simulink model "IEEE123bus_v2019b_Phasor_DPL_ZIPload"  (R2019b)
settings: Solver=VariableStepAuto  StartTime=0.0  StopTime=100  FixedStep=Ts  RelTol=1e-3
InitFcn:
  | a=1; % Loading Factor
  | Ts=0.1;% For Delay Blocks in Voltage Regulator Controls
  | 
  | % Simulation data for the IEEE 123 Node Test Feeder model
  | mi2km = 1.60934;%  miles to km conversion
  | ft2km = 0.0003048; % feet to km conversion
  | ms2F = 1*1e-6/(2*pi*60);% microsiemens to Farads conversion
  | 
  | %% Configuration 1
  | % Series Resitance and Reactance - ohm/mile
  | R_1 = [0.4576 0.1560 0.1535;0.1560 0.4666 0.1580;0.1535 0.1580 0.4615];
  | X_1 = [1.0780 0.5017 0.3849;0.5017 1.0482 0.4236;0.3849 0.4236 1.0651];
  | % charging susceptance - microsiemens/mile
  | B_1 = [5.6765 -1.8319 -0.6982;-1.8319 5.9809 -1.1645;-0.6982 -1.1645 5.3971];
  | 
  | R_1 = R_1/mi2km;
  | L_1 = (X_1/(2*pi*60))/mi2km;
  | C_1 =(B_1*ms2F)/mi2km;
  | 
  | %% Configuration 2 - series reactance - ohm/mile
  | R_2 = [0.4666 0.1580 0.1560;0.1580 0.4615 0.1535;0.1560 0.1535 0.4576];
  | X_2 = [1.0482 0.4236 0.5017;0.4236 1.0651 0.3849;0.5017 0.3849 1.0780];
  | % charging susceptance - microsiemens/mile
  | B_2 = [5.9809 -1.1645 -1.8319;-1.1645 5.3971 -0.6982;-1.8319 -0.6982 5.6765];
  | 
  | R_2 = R_2/mi2km;
  | L_2 = (X_2/(2*pi*60))/mi2km;
  | C_2 =(B_2*ms2F)/mi2km;
  | 
  | %% Configuration 3 - series reactance - ohm/mile
  | R_3 = [0.4615 0.1535 0.1580;0.1535 0.4576 0.1560;0.1580 0.1560 0.4666];
  | X_3 = [1.0651 0.3849 0.4236;0.3849 1.0780 0.5017;0.4236 0.5017 1.0482];
  | % charging susceptance - microsiemens/mile
  | B_3 = [5.3971 -0.6982 -1.1645;-0.6982 5.6765 -1.8319; -1.1645 -1.8319 5.9809];
  | 
  | R_3 = R_3/mi2km;
  | L_3 = (X_3/(2*pi*60))/mi2km;
  | C_3 =(B_3*ms2F)/mi2km;
  | 
  | %% Configuration 4 - series reactance - ohm/mile
  | R_4 = [0.4615 0.1580 0.1535;0.1580 0.4666 0.1560;0.1535 0.1560 0.4576];
  | X_4 = [1.0651 0.4236 0.3849;0.4236 1.0482 0.5017;0.3849 0.5017 1.0780];
  | % charging susceptance - microsiemens/mile
  | B_4 = [5.3971 -1.1645 -0.6982;-1.1645 5.9809 -1.8319;-0.6982 -1.8319 5.6765];
  | 
  | R_4 = R_4/mi2km;
  | L_4 = (X_4/(2*pi*60))/mi2km;
  | C_4 =(B_4*ms2F)/mi2km;
  | 
  | %% Configuration 5 - series reactance - ohm/mile
  | R_5 = [0.4666 0.1560 0.1580;0.1560 0.4576 0.1535;0.1580 0.1535 0.4615];
  | X_5 = [1.0482 0.5017 0.4236;0.5017 1.0780 0.3849;0.4236 0.3849 1.0651];
  | % charging susceptance - microsiemens/mile
  | B_5 = [5.9809 -1.8319 -1.1645;-1.8319 5.6765 -0.6982;-1.1645 -0.6982 5.3971];
  | 
  | R_5 = R_5/mi2km;
  | L_5 = (X_5/(2*pi*60))/mi2km;
  | C_5 =(B_5*ms2F)/mi2km;
  | 
  | %% Configuration 6 - series reactance - ohm/mile
  | R_6 = [0.4576 0.1535 0.1560;0.1535 0.4615 0.1580;0.1560 0.1580 0.4666];
  | X_6 = [1.0780 0.3849 0.5017;0.3849 1.0651 0.4236;0.5017 0.4236 1.0482];
  | % charging susceptance - microsiemens/mile
  | B_6 = [5.6765 -0.6982 -1.8319;-0.6982 5.3971 -1.1645;-1.8319 -1.1645 5.9809];
  | 
  | R_6 = R_6/mi2km;
  | L_6 = (X_6/(2*pi*60))/mi2km;
  | C_6 =(B_6*ms2F)/mi2km;
  | 
  | %% Configuration 7 - series reactance - ohm/mile
  | R_7 = [0.4576 0.0000 0.1535;0.0000 0.0000 0.0000;0.1535 0.0000 0.4615];
  | X_7 = [1.0780 0.0000 0.3849;0.0000 0.0000 0.0000;0.3849 0.0000 1.0651];
  | % charging susceptance - microsiemens/mile
  | B_7 = [5.1154 0.0000 -1.0549;0.0000 0.0000 0.0000;-1.0549 0.0000 5.1704];
  | 
  | R_7 = R_7/mi2km;
  | L_7 = (X_7/(2*pi*60))/mi2km;
  | C_7 =(B_7*ms2F)/mi2km;
  | 
  | %% Configuration 8 - series reactance - ohm/mile
  | R_8 = [0.4576 0.1535 0.0000;0.1535 0.4615 0.0000;0.0000 0.0000 0.0000];
  | X_8 = [1.0780 0.3849 0.0000;0.3849 1.0651 0.0000;0.0000 0.0000 0.0000];
  | % charging susceptance - microsiemens/mile
  | B_8 = [5.1154 -1.0549 0.0000;-1.0549 5.1704 0.0000;0.0000 0.0000 0.0000];
  | 
  | R_8 = R_8/mi2km;
  | L_8 = (X_8/(2*pi*60))/mi2km;
  | C_8 =(B_8*ms2F)/mi2km;
  | 
  | %% Configuration 9 - series reactance - ohm/mile
  | R_9 = [1.3292 0 0;0 0 0;0 0 0];
  | X_9 = [1.3475 0 0;0 0 0;0 0 0];
  | % charging susceptance - microsiemens/mile
  | B_9 = [4.5193 0 0;0 0 0;0 0 0];
  | 
  | R_9 = R_9/mi2km;
  | L_9 = (X_9/(2*pi*60))/mi2km;
  | C_9 =(B_9*ms2F)/mi2km;
  | 
  | %% Configuration 10- series reactance - ohm/mile
  | R_10 = [0 0 0;0 1.3292 0;0 0 0];
  | X_10 = [0 0 0;0 1.3475 0;0 0 0];
  | % charging susceptance - microsiemens/mile
  | B_10 = [0 0 0;0 4.5193 0;0 0 0];
  | 
  | R_10 = R_10/mi2km;
  | L_10 = (X_10/(2*pi*60))/mi2km;
  | C_10 =(B_10*ms2F)/mi2km;
  | 
  | %% Configuration 11 - series reactance - ohm/mile
  | R_11 = [0 0 0;0 0 0;0 0 1.3292];
  | X_11 = [0 0 0;0 0 0;0 0 1.3475];
  | % charging susceptance - microsiemens/mile
  | B_11 = [0 0 0;0 0 0;0 0 4.5193];
  | 
  | R_11 = R_11/mi2km;
  | L_11 = (X_11/(2*pi*60))/mi2km;
  | C_11 =(B_11*ms2F)/mi2km;
  | 
  | %% Configuration 12 - series reactance - ohm/mile
  | R_12 = [1.5209 0.5198 0.4924;0.5198 1.5329 0.5198;0.4924 0.5198 1.5209];
  | X_12 = [0.7521 0.2775 0.2157;0.2775 0.7162 0.2775;0.2157 0.2775 0.7521];
  | % charging susceptance - microsiemens/mile
  | B_12 = [67.2242 0.0000 0.0000;0.0000 67.2242 0.0000;0.0000 0.0000 67.2242];
  | 
  | R_12 = R_12/mi2km;
  | L_12 = (X_12/(2*pi*60))/mi2km;
  | C_12 =(B_12*ms2F)/mi2km;
undefined symbols (not defined in the file or in its folder): D1, Delta, find_system, j
libraries: powerlib x886, powerlib_meascontrol x31
(part 1 of 12)
settings Model: ARTEMISmethode_block_infos=$$__separator__$$pi123variableloadwith3PV/ARTEMIS Guide$$__separator__$$  Creator=Arun  LastModifiedBy=USARSUR
settings DataIOCC: ReturnWorkspaceOutputs=off
settings DebuggingCC: UnconnectedInputMsg=none  UnconnectedOutputMsg=none  UnconnectedLineMsg=none  ArithmeticOperatorsInVariantConditions=warning
settings SFSimCC: SimUseLocalCustomCode=off  CustomCodeUndefinedFunction=UseInterfaceOnly
settings RTWCC: RTWUseLocalCustomCode=off
settings CodeAppCC: StateflowObjectComments=on
settings SimscapeCC: SimscapeNormalizeSystem=off

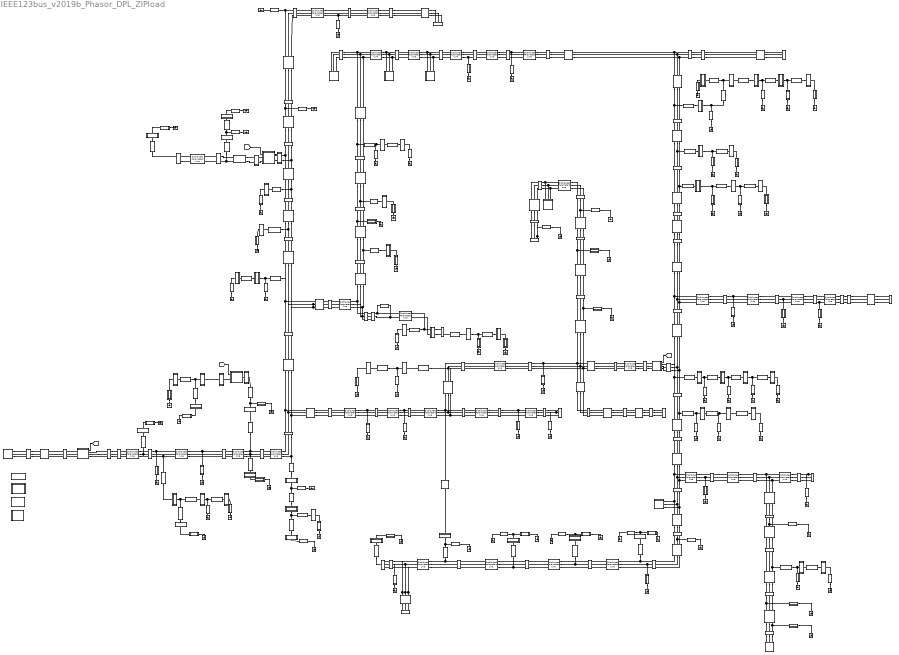
== system IEEE123bus_v2019b_Phasor_DPL_ZIPload ==
  note: Please consider citing following papers if the model was useful for your research
      |
      | A. Suresh, R. Bisht and S. Kamalasadan, "A Coordinated Control Architecture With Inverter-Based Resources and Legacy
      | Controllers of Power Distribution System for Voltage Profile Balance," in IEEE Transactions on Industry Applications, vol. 58,
      | no. 5, pp. 6701-6712, Sept.-Oct. 2022, doi: 10.1109/TIA.2022.3183030.
      |
      | A. Suresh, R. Bisht and S. Kamalasadan, "ADMM Based LQR for Voltage Regulation Using Distributed Energy Resources,"
      | 2020 IEEE International Conference on Power Electronics, Drives and Energy Systems (PEDES), 2020, pp. 1-6,
      | doi: 10.1109/PEDES49360.2020.9379625.
  note: Model Developed by
      | Arun Suresh, Dr. Sukumar Kamalasadan,
      | University of North Carolina, Charlotte
  1 : powerlib/Measurements/Three-Phase V-I Measurement  VoltageMeasurement=phase-to-ground  SetLabelV=on  LabelV=V1  Vpu=off  VpuLL=off  CurrentMeasurement=no  SetLabelI=on  LabelI=I800  Ipu=off  Pbase=100e6  Vbase=24900  OutputType=Complex  PhasorSimulation=on  PSBequivalent=0
      settings: SourceProductName=Simscape Electrical
  1 Y PQ : Subsystem  mask(Single Phase ZIP Load){Vnom=1.0*2401.78, fnom=60, Pnom=40e3*a, Qnom=20e3*a, LoadType=constant P, Vlim=0.7}
      mask prompts: Vnom "Nominal Voltage Vn (Vrms)"; fnom "Nominal Frequency fn (Hz)"; Pnom "Nominal Active power (W)"; Qnom "Nominal Reactive power (VAR)"; LoadType "Load Type"; Vlim "Minimum voltage (pu)"
      mask help:
      | Notes:
      | Single Phase ZIP load model which gets converted to constant Z type if the voltage becomes lower than the Minimum Voltage.
      mask TypeOptions LoadType: Constant Z | constant I | constant P
      mask DialogControl ParameterTabVar0 Prompt: Parameters
      mask DialogControl ParameterTabVar1 Prompt: Type
      mask Display:
      | color('red');
      | A=[-210,-180,-170,-160,-147,-140,-130,-120,-110,-80,-50,-49,-45,-39,-33,-26,-21,-18,-17,-19,-22,-22,-26,-27,-25,-22,-16,-9,-3,2,6,6,4,1,1,-3,-4,-2,2,7,14,20,26,29,30,28,24,24,21,20,21,25,31,37,44,49,50,50,80];
      | B=[-41.5,-41.5,-63,-20,-63,-20,-63,-20,-41.5,-41.5,-41.5,-34,-26,-21,-20,-22,-28,-37,-47,-57,-63,-63,-54,-44,-34,-26,-21,-20,-22,-28,-37,-47,-57,-63,-63,-54,-44,-34,-26,-21,-20,-22,-28,-37,-47,-57,-63,-63,-54,-44,-34,-26,-21,-20,-22,-28,-37,-41.50,-41.5];
      | plot(A,B);
      | color('black');
      | port_label('LConn', 1, '+')
  1-2 10 : powerlib/Elements/Distributed Parameters Line  Phases=1  Frequency=60  Resistance=R_10(2,2)  Inductance=L_10(2,2)  Capacitance=C_10(2,2)  Length=175*ft2km  x1=[3403.40407583669;376.991118430775;-2.09535227015144]  x2=[3403.40393728209;376.991118430775;-2.09535231811345]  x3=[6.22904140851351;376.991118430775;-2.09543411070126]  x4=[6.2358477770861;376.991118430775;-2.09535231481402]  x5=2.16957196133287e-07  V1=[2.049e+04;377;-2.115]  V2=[2.048e+04;377;-2.115]  I1=[33.62;377;-2.106]  I2=[35.2;377;-2.126]  nHarmo=1  Measurements=None
      settings: SourceProductName=Simscape Electrical
  1-3 11 : powerlib/Elements/Distributed Parameters Line  Phases=1  Frequency=60  Resistance=R_11(3,3)  Inductance=L_11(3,3)  Capacitance=C_11(3,3)  Length=250*ft2km  x1=[3404.23228446094;376.991118430775;2.09338339619212]  x2=[3404.23180903077;376.991118430775;2.09338315630066]  x3=[6.22358820978929;376.991118430775;2.09290352483269]  x4=[6.24401143477824;376.991118430775;2.09374480200052]  x5=3.09938851618982e-07  V1=[2.049e+04;377;-2.115]  V2=[2.048e+04;377;-2.115]  I1=[33.62;377;-2.106]  I2=[35.2;377;-2.126]  nHarmo=1  Measurements=None
      settings: SourceProductName=Simscape Electrical
  1-7 1 : powerlib/Elements/Distributed Parameters Line  Phases=3  Frequency=60  Resistance=R_1  Inductance=L_1  Capacitance=C_1  Length=300*ft2km  x1=[436.800297543745 4167.29457653455 4166.80094747361;376.991118430775 376.991118430775 376.991118430775;1.69106599673736 -2.40312878788664 2.3092308326774]  x2=[437.061191479492 4173.08837477824 4174.13245807205;376.991118430775 376.991118430775 376.991118430775;1.69067039189404 -2.40392213512409 2.30843926486521]  x3=[2.63602464413822 185.698581223299 185.612678797795;376.991118430775 376.991118430775 376.991118430775;0.131396490934745 2.37819332141936 0.79306646276384]  x4=[2.86335918238174 186.149188672012 185.887033927544;376.991118430775 376.991118430775 376.991118430775;2.8602728168382 -0.931024482265744 -2.48097001414768]  x5=3.76244991844366e-07  V1=ones(3,3)  V2=ones(3,3)  I1=ones(3,3)  I2=ones(3,3)  nHarmo=1  Measurements=None
      settings: SourceProductName=Simscape Electrical
  10 : Subsystem
  10 Y I : Subsystem  mask(Single Phase ZIP Load){Vnom=1.0*2401.78, fnom=60, Pnom=20e3*a, Qnom=10e3*a, LoadType=constant I, Vlim=0.7}
      mask prompts: Vnom "Nominal Voltage Vn (Vrms)"; fnom "Nominal Frequency fn (Hz)"; Pnom "Nominal Active power (W)"; Qnom "Nominal Reactive power (VAR)"; LoadType "Load Type"; Vlim "Minimum voltage (pu)"
      mask help:
      | Notes:
      | Single Phase ZIP load model which gets converted to constant Z type if the voltage becomes lower than the Minimum Voltage.
      mask TypeOptions LoadType: Constant Z | constant I | constant P
      mask DialogControl ParameterTabVar0 Prompt: Parameters
      mask DialogControl ParameterTabVar1 Prompt: Type
      mask Display:
      | color('red');
      | A=[-210,-180,-170,-160,-147,-140,-130,-120,-110,-80,-50,-49,-45,-39,-33,-26,-21,-18,-17,-19,-22,-22,-26,-27,-25,-22,-16,-9,-3,2,6,6,4,1,1,-3,-4,-2,2,7,14,20,26,29,30,28,24,24,21,20,21,25,31,37,44,49,50,50,80];
      | B=[-41.5,-41.5,-63,-20,-63,-20,-63,-20,-41.5,-41.5,-41.5,-34,-26,-21,-20,-22,-28,-37,-47,-57,-63,-63,-54,-44,-34,-26,-21,-20,-22,-28,-37,-47,-57,-63,-63,-54,-44,-34,-26,-21,-20,-22,-28,-37,-47,-57,-63,-63,-54,-44,-34,-26,-21,-20,-22,-28,-37,-41.50,-41.5];
      | plot(A,B);
      | color('black');
      | port_label('LConn', 1, '+')
  100 : powerlib/Measurements/Three-Phase V-I Measurement  VoltageMeasurement=phase-to-ground  SetLabelV=on  LabelV=V100  Vpu=off  VpuLL=off  CurrentMeasurement=no  SetLabelI=on  LabelI=I65  Ipu=off  Pbase=100e6  Vbase=24900  OutputType=Complex  PhasorSimulation=on  PSBequivalent=0
      settings: SourceProductName=Simscape Electrical
  100 Y Z : Subsystem  mask(Single Phase ZIP Load){Vnom=1.0*2401.78, fnom=60, Pnom=40e3*a, Qnom=20e3*a, LoadType=Constant Z, Vlim=0.7}
      mask prompts: Vnom "Nominal Voltage Vn (Vrms)"; fnom "Nominal Frequency fn (Hz)"; Pnom "Nominal Active power (W)"; Qnom "Nominal Reactive power (VAR)"; LoadType "Load Type"; Vlim "Minimum voltage (pu)"
      mask help:
      | Notes:
      | Single Phase ZIP load model which gets converted to constant Z type if the voltage becomes lower than the Minimum Voltage.
      mask TypeOptions LoadType: Constant Z | constant I | constant P
      mask DialogControl ParameterTabVar0 Prompt: Parameters
      mask DialogControl ParameterTabVar1 Prompt: Type
      mask Display:
      | color('red');
      | A=[-210,-180,-170,-160,-147,-140,-130,-120,-110,-80,-50,-49,-45,-39,-33,-26,-21,-18,-17,-19,-22,-22,-26,-27,-25,-22,-16,-9,-3,2,6,6,4,1,1,-3,-4,-2,2,7,14,20,26,29,30,28,24,24,21,20,21,25,31,37,44,49,50,50,80];
      | B=[-41.5,-41.5,-63,-20,-63,-20,-63,-20,-41.5,-41.5,-41.5,-34,-26,-21,-20,-22,-28,-37,-47,-57,-63,-63,-54,-44,-34,-26,-21,-20,-22,-28,-37,-47,-57,-63,-63,-54,-44,-34,-26,-21,-20,-22,-28,-37,-47,-57,-63,-63,-54,-44,-34,-26,-21,-20,-22,-28,-37,-41.50,-41.5];
      | plot(A,B);
      | color('black');
      | port_label('LConn', 1, '+')
  100-450 3 : powerlib/Elements/Distributed Parameters Line  Phases=3  Frequency=60  Resistance=R_3  Inductance=L_3  Capacitance=C_3  Length=800*ft2km  x1=[443.373552146088 4232.26022753008 4232.1634537403;376.991118430775 376.991118430775 376.991118430775;-0.417224791555343 0.205878059890174 1.77874707649804]  x2=[443.373583862276 4232.26043412699 4232.16366214147;376.991118430775 376.991118430775 376.991118430775;-0.417224820253187 0.20587803856342 1.77874704932021]  x3=[0.582709365484829 12.4738244359709 15.7961847761454;376.991118430775 376.991118430775 376.991118430775;-0.417603048631578 0.205565591892628 1.77843324057499]  x4=[0.582709365503137 12.4738244359882 15.7961847761854;376.991118430775 376.991118430775 376.991118430775;-0.417224820241726 0.205878038563425 1.7787470493196]  x5=1.00331997825164e-06  V1=ones(3,3)  V2=ones(3,3)  I1=ones(3,3)  I2=ones(3,3)  nHarmo=1  Measurements=None
      settings: SourceProductName=Simscape Electrical
  101 : powerlib/Measurements/Three-Phase V-I Measurement  VoltageMeasurement=phase-to-ground  SetLabelV=on  LabelV=V101  Vpu=off  VpuLL=off  CurrentMeasurement=no  SetLabelI=on  LabelI=I65  Ipu=off  Pbase=100e6  Vbase=24900  OutputType=Complex  PhasorSimulation=on  PSBequivalent=0
      settings: SourceProductName=Simscape Electrical
  101-102 11 : powerlib/Elements/Distributed Parameters Line  Phases=1  Frequency=60  Resistance=R_11(3,3)  Inductance=L_11(3,3)  Capacitance=C_11(3,3)  Length=225*ft2km  x1=[3457.92797170476;376.991118430775;2.08694980209931]  x2=[3457.92757743413;376.991118430775;2.08694957468531]  x3=[6.32180933144979;376.991118430775;2.08636460802156]  x4=[6.3425547416883;376.991118430775;2.08742786454813]  x5=2.78944966457084e-07  V1=[2.049e+04;377;-2.115]  V2=[2.048e+04;377;-2.115]  I1=[33.62;377;-2.106]  I2=[35.2;377;-2.126]  nHarmo=1  Measurements=None
      settings: SourceProductName=Simscape Electrical
  101-105 3 : powerlib/Elements/Distributed Parameters Line  Phases=3  Frequency=60  Resistance=R_3  Inductance=L_3  Capacitance=C_3  Length=275*ft2km  x1=[443.373660115841 4232.25950788553 4232.16299468928;376.991118430775 376.991118430775 376.991118430775;-0.416978675467481 0.206083103238666 1.77895313392089]  x2=[443.374129264306 4232.25962050144 4232.16326999734;376.991118430775 376.991118430775 376.991118430775;-0.416979795125428 0.206082912265049 1.77895300387884]  x3=[0.580098762037406 12.4571733375896 15.786970190557;376.991118430775 376.991118430775 376.991118430775;-0.427075702485888 0.20516777463084 1.77792629805874]  x4=[0.585465938762827 12.4921559124847 15.8081037031614;376.991118430775 376.991118430775 376.991118430775;-0.407104755765716 0.206888419808551 1.77987066114847]  x5=3.44891242524002e-07  V1=ones(3,3)  V2=ones(3,3)  I1=ones(3,3)  I2=ones(3,3)  nHarmo=1  Measurements=None
      settings: SourceProductName=Simscape Electrical
  102 : Subsystem
  102 Y PQ : Subsystem  mask(Single Phase ZIP Load){Vnom=1.0*2401.78, fnom=60, Pnom=20e3*a, Qnom=10e3*a, LoadType=constant P, Vlim=0.7}
      mask prompts: Vnom "Nominal Voltage Vn (Vrms)"; fnom "Nominal Frequency fn (Hz)"; Pnom "Nominal Active power (W)"; Qnom "Nominal Reactive power (VAR)"; LoadType "Load Type"; Vlim "Minimum voltage (pu)"
      mask help:
      | Notes:
      | Single Phase ZIP load model which gets converted to constant Z type if the voltage becomes lower than the Minimum Voltage.
      mask TypeOptions LoadType: Constant Z | constant I | constant P
      mask DialogControl ParameterTabVar0 Prompt: Parameters
      mask DialogControl ParameterTabVar1 Prompt: Type
      mask Display:
      | color('red');
      | A=[-210,-180,-170,-160,-147,-140,-130,-120,-110,-80,-50,-49,-45,-39,-33,-26,-21,-18,-17,-19,-22,-22,-26,-27,-25,-22,-16,-9,-3,2,6,6,4,1,1,-3,-4,-2,2,7,14,20,26,29,30,28,24,24,21,20,21,25,31,37,44,49,50,50,80];
      | B=[-41.5,-41.5,-63,-20,-63,-20,-63,-20,-41.5,-41.5,-41.5,-34,-26,-21,-20,-22,-28,-37,-47,-57,-63,-63,-54,-44,-34,-26,-21,-20,-22,-28,-37,-47,-57,-63,-63,-54,-44,-34,-26,-21,-20,-22,-28,-37,-47,-57,-63,-63,-54,-44,-34,-26,-21,-20,-22,-28,-37,-41.50,-41.5];
      | plot(A,B);
      | color('black');
      | port_label('LConn', 1, '+')
  102-103 11 : powerlib/Elements/Distributed Parameters Line  Phases=1  Frequency=60  Resistance=R_11(3,3)  Inductance=L_11(3,3)  Capacitance=C_11(3,3)  Length=325*ft2km  x1=[3457.92757743413;376.991118430775;2.08690283700759]  x2=[3457.92722333804;376.991118430775;2.08690261072161]  x3=[6.32504721964269;376.991118430775;2.08642323448268]  x4=[6.33887685523373;376.991118430775;2.08722942969897]  x5=4.02920507104677e-07  V1=[2.049e+04;377;-2.115]  V2=[2.048e+04;377;-2.115]  I1=[33.62;377;-2.106]  I2=[35.2;377;-2.126]  nHarmo=1  Measurements=None
      settings: SourceProductName=Simscape Electrical
  103 : Subsystem
  103 Y PQ : Subsystem  mask(Single Phase ZIP Load){Vnom=1.0*2401.78, fnom=60, Pnom=40e3*a, Qnom=20e3*a, LoadType=constant P, Vlim=0.7}
      mask prompts: Vnom "Nominal Voltage Vn (Vrms)"; fnom "Nominal Frequency fn (Hz)"; Pnom "Nominal Active power (W)"; Qnom "Nominal Reactive power (VAR)"; LoadType "Load Type"; Vlim "Minimum voltage (pu)"
      mask help:
      | Notes:
      | Single Phase ZIP load model which gets converted to constant Z type if the voltage becomes lower than the Minimum Voltage.
      mask TypeOptions LoadType: Constant Z | constant I | constant P
      mask DialogControl ParameterTabVar0 Prompt: Parameters
      mask DialogControl ParameterTabVar1 Prompt: Type
      mask Display:
      | color('red');
      | A=[-210,-180,-170,-160,-147,-140,-130,-120,-110,-80,-50,-49,-45,-39,-33,-26,-21,-18,-17,-19,-22,-22,-26,-27,-25,-22,-16,-9,-3,2,6,6,4,1,1,-3,-4,-2,2,7,14,20,26,29,30,28,24,24,21,20,21,25,31,37,44,49,50,50,80];
      | B=[-41.5,-41.5,-63,-20,-63,-20,-63,-20,-41.5,-41.5,-41.5,-34,-26,-21,-20,-22,-28,-37,-47,-57,-63,-63,-54,-44,-34,-26,-21,-20,-22,-28,-37,-47,-57,-63,-63,-54,-44,-34,-26,-21,-20,-22,-28,-37,-47,-57,-63,-63,-54,-44,-34,-26,-21,-20,-22,-28,-37,-41.50,-41.5];
      | plot(A,B);
      | color('black');
      | port_label('LConn', 1, '+')
  103-104 11 : powerlib/Elements/Distributed Parameters Line  Phases=1  Frequency=60  Resistance=R_11(3,3)  Inductance=L_11(3,3)  Capacitance=C_11(3,3)  Length=700*ft2km  x1=[3457.92722333804;376.991118430775;2.08672734443013]  x2=[3457.92679904314;376.991118430775;2.08672711299265]  x3=[6.32768318900497;376.991118430775;2.08639997569265]  x4=[6.33459681116843;376.991118430775;2.08672711297322]  x5=8.6782878453315e-07  V1=[2.049e+04;377;-2.115]  V2=[2.048e+04;377;-2.115]  I1=[33.62;377;-2.106]  I2=[35.2;377;-2.126]  nHarmo=1  Measurements=None
      settings: SourceProductName=Simscape Electrical
  104 : Subsystem
  104 Y PQ : Subsystem  mask(Single Phase ZIP Load){Vnom=1.0*2401.78, fnom=60, Pnom=40e3*a, Qnom=20e3*a, LoadType=constant P, Vlim=0.7}
      mask prompts: Vnom "Nominal Voltage Vn (Vrms)"; fnom "Nominal Frequency fn (Hz)"; Pnom "Nominal Active power (W)"; Qnom "Nominal Reactive power (VAR)"; LoadType "Load Type"; Vlim "Minimum voltage (pu)"
      mask help:
      | Notes:
      | Single Phase ZIP load model which gets converted to constant Z type if the voltage becomes lower than the Minimum Voltage.
      mask TypeOptions LoadType: Constant Z | constant I | constant P
      mask DialogControl ParameterTabVar0 Prompt: Parameters
      mask DialogControl ParameterTabVar1 Prompt: Type
      mask Display:
      | color('red');
      | A=[-210,-180,-170,-160,-147,-140,-130,-120,-110,-80,-50,-49,-45,-39,-33,-26,-21,-18,-17,-19,-22,-22,-26,-27,-25,-22,-16,-9,-3,2,6,6,4,1,1,-3,-4,-2,2,7,14,20,26,29,30,28,24,24,21,20,21,25,31,37,44,49,50,50,80];
      | B=[-41.5,-41.5,-63,-20,-63,-20,-63,-20,-41.5,-41.5,-41.5,-34,-26,-21,-20,-22,-28,-37,-47,-57,-63,-63,-54,-44,-34,-26,-21,-20,-22,-28,-37,-47,-57,-63,-63,-54,-44,-34,-26,-21,-20,-22,-28,-37,-47,-57,-63,-63,-54,-44,-34,-26,-21,-20,-22,-28,-37,-41.50,-41.5];
      | plot(A,B);
      | color('black');
      | port_label('LConn', 1, '+')
  105 : powerlib/Measurements/Three-Phase V-I Measurement  VoltageMeasurement=phase-to-ground  SetLabelV=on  LabelV=V105  Vpu=off  VpuLL=off  CurrentMeasurement=no  SetLabelI=on  LabelI=I65  Ipu=off  Pbase=100e6  Vbase=24900  OutputType=Complex  PhasorSimulation=on  PSBequivalent=0
      settings: SourceProductName=Simscape Electrical
  105-106 10 : powerlib/Elements/Distributed Parameters Line  Phases=1  Frequency=60  Resistance=R_10(2,2)  Inductance=L_10(2,2)  Capacitance=C_10(2,2)  Length=225*ft2km  x1=[3454.84642633286;376.991118430775;-2.10369664777796]  x2=[3454.84615169221;376.991118430775;-2.10369679595318]  x3=[6.3196296545121;376.991118430775;-2.1040709672509]  x4=[6.33344760701491;376.991118430775;-2.10342834076941]  x5=2.78944966457084e-07  V1=[2.049e+04;377;-2.115]  V2=[2.048e+04;377;-2.115]  I1=[33.62;377;-2.106]  I2=[35.2;377;-2.126]  nHarmo=1  Measurements=None
      settings: SourceProductName=Simscape Electrical
  105-108 3 : powerlib/Elements/Distributed Parameters Line  Phases=3  Frequency=60  Resistance=R_3  Inductance=L_3  Capacitance=C_3  Length=325*ft2km  x1=[443.374129264306 4232.25962050144 4232.16326999734;376.991118430775 376.991118430775 376.991118430775;-0.417003435295474 0.20606338368171 1.77893338998289]  x2=[443.374706647336 4232.25969906192 4232.16360921195;376.991118430775 376.991118430775 376.991118430775;-0.417006345127648 0.206063208765789 1.7789333495239]  x3=[0.575007685408612 12.4608177468437 15.7977642338539;376.991118430775 376.991118430775 376.991118430775;-0.431112090174094 0.205370810020635 1.77825349855094]  x4=[0.590603688952939 12.4883481256447 15.7970465206151;376.991118430775 376.991118430775 376.991118430775;-0.403421875407038 0.206627458212945 1.77948577638124]  x5=4.0759874116473e-07  V1=ones(3,3)  V2=ones(3,3)  I1=ones(3,3)  I2=ones(3,3)  nHarmo=1  Measurements=None
      settings: SourceProductName=Simscape Electrical
  106 : Subsystem
  106 Y PQ : Subsystem  mask(Single Phase ZIP Load){Vnom=1.0*2401.78, fnom=60, Pnom=40e3*a, Qnom=20e3*a, LoadType=constant P, Vlim=0.7}
      mask prompts: Vnom "Nominal Voltage Vn (Vrms)"; fnom "Nominal Frequency fn (Hz)"; Pnom "Nominal Active power (W)"; Qnom "Nominal Reactive power (VAR)"; LoadType "Load Type"; Vlim "Minimum voltage (pu)"
      mask help:
      | Notes:
      | Single Phase ZIP load model which gets converted to constant Z type if the voltage becomes lower than the Minimum Voltage.
      mask TypeOptions LoadType: Constant Z | constant I | constant P
      mask DialogControl ParameterTabVar0 Prompt: Parameters
      mask DialogControl ParameterTabVar1 Prompt: Type
      mask Display:
      | color('red');
      | A=[-210,-180,-170,-160,-147,-140,-130,-120,-110,-80,-50,-49,-45,-39,-33,-26,-21,-18,-17,-19,-22,-22,-26,-27,-25,-22,-16,-9,-3,2,6,6,4,1,1,-3,-4,-2,2,7,14,20,26,29,30,28,24,24,21,20,21,25,31,37,44,49,50,50,80];
      | B=[-41.5,-41.5,-63,-20,-63,-20,-63,-20,-41.5,-41.5,-41.5,-34,-26,-21,-20,-22,-28,-37,-47,-57,-63,-63,-54,-44,-34,-26,-21,-20,-22,-28,-37,-47,-57,-63,-63,-54,-44,-34,-26,-21,-20,-22,-28,-37,-47,-57,-63,-63,-54,-44,-34,-26,-21,-20,-22,-28,-37,-41.50,-41.5];
      | plot(A,B);
      | color('black');
      | port_label('LConn', 1, '+')
  106-107 10 : powerlib/Elements/Distributed Parameters Line  Phases=1  Frequency=60  Resistance=R_10(2,2)  Inductance=L_10(2,2)  Capacitance=C_10(2,2)  Length=575*ft2km  x1=[3454.84615169221;376.991118430775;-2.10386037782523]  x2=[3454.84577635343;376.991118430775;-2.10386056019097]  x3=[6.32231830333193;376.991118430775;-2.1041292839401]  x4=[6.32922616371457;376.991118430775;-2.1038605602597]  x5=7.12859358723659e-07  V1=[2.049e+04;377;-2.115]  V2=[2.048e+04;377;-2.115]  I1=[33.62;377;-2.106]  I2=[35.2;377;-2.126]  nHarmo=1  Measurements=None
      settings: SourceProductName=Simscape Electrical
  107 : Subsystem
  107 Y PQ : Subsystem  mask(Single Phase ZIP Load){Vnom=1.0*2401.78, fnom=60, Pnom=40e3*a, Qnom=20e3*a, LoadType=constant P, Vlim=0.7}
      mask prompts: Vnom "Nominal Voltage Vn (Vrms)"; fnom "Nominal Frequency fn (Hz)"; Pnom "Nominal Active power (W)"; Qnom "Nominal Reactive power (VAR)"; LoadType "Load Type"; Vlim "Minimum voltage (pu)"
      mask help:
      | Notes:
      | Single Phase ZIP load model which gets converted to constant Z type if the voltage becomes lower than the Minimum Voltage.
      mask TypeOptions LoadType: Constant Z | constant I | constant P
      mask DialogControl ParameterTabVar0 Prompt: Parameters
      mask DialogControl ParameterTabVar1 Prompt: Type
      mask Display:
      | color('red');
      | A=[-210,-180,-170,-160,-147,-140,-130,-120,-110,-80,-50,-49,-45,-39,-33,-26,-21,-18,-17,-19,-22,-22,-26,-27,-25,-22,-16,-9,-3,2,6,6,4,1,1,-3,-4,-2,2,7,14,20,26,29,30,28,24,24,21,20,21,25,31,37,44,49,50,50,80];
      | B=[-41.5,-41.5,-63,-20,-63,-20,-63,-20,-41.5,-41.5,-41.5,-34,-26,-21,-20,-22,-28,-37,-47,-57,-63,-63,-54,-44,-34,-26,-21,-20,-22,-28,-37,-47,-57,-63,-63,-54,-44,-34,-26,-21,-20,-22,-28,-37,-47,-57,-63,-63,-54,-44,-34,-26,-21,-20,-22,-28,-37,-41.50,-41.5];
      | plot(A,B);
      | color('black');
      | port_label('LConn', 1, '+')
  108 : powerlib/Measurements/Three-Phase V-I Measurement  VoltageMeasurement=phase-to-ground  SetLabelV=on  LabelV=V108  Vpu=off  VpuLL=off  CurrentMeasurement=no  SetLabelI=on  LabelI=I65  Ipu=off  Pbase=100e6  Vbase=24900  OutputType=Complex  PhasorSimulation=on  PSBequivalent=0
      settings: SourceProductName=Simscape Electrical
  108-109 9 : powerlib/Elements/Distributed Parameters Line  Phases=1  Frequency=60  Resistance=R_9(1,1)  Inductance=L_9(1,1)  Capacitance=C_9(1,1)  Length=450*ft2km  x1=[3458.20538432056;376.991118430775;-0.0100922145782953]  x2=[3458.20413088381;376.991118430775;-0.0100929899969072]  x3=[6.31491128604917;376.991118430775;-0.0111701752884377]  x4=[6.34948613236906;376.991118430775;-0.00923065479675195]  x5=5.57889932914168e-07  V1=[2.049e+04;377;-2.115]  V2=[2.048e+04;377;-2.115]  I1=[33.62;377;-2.106]  I2=[35.2;377;-2.126]  nHarmo=1  Measurements=None
      settings: SourceProductName=Simscape Electrical
  108-300 3 : powerlib/Elements/Distributed Parameters Line  Phases=3  Frequency=60  Resistance=R_3  Inductance=L_3  Capacitance=C_3  Length=1000*ft2km  x1=[443.374706647336 4232.25969906192 4232.16360921195;376.991118430775 376.991118430775 376.991118430775;-0.417325487423277 0.205799572890717 1.77866856192854]  x2=[443.374756007601 4232.26001559536 4232.163929932;376.991118430775 376.991118430775 376.991118430775;-0.417325530868192 0.205799538322098 1.77866851864881]  x3=[0.582695619827279 12.4734531696118 15.795627917319;376.991118430775 376.991118430775 376.991118430775;-0.417796485158491 0.205411000377545 1.77827764894123]  x4=[0.58269303451633 12.4735547103566 15.7957176842165;376.991118430775 376.991118430775 376.991118430775;-0.417327357905288 0.20579752093348 1.77866713137837]  x5=1.25414997281455e-06  V1=ones(3,3)  V2=ones(3,3)  I1=ones(3,3)  I2=ones(3,3)  nHarmo=1  Measurements=None
      settings: SourceProductName=Simscape Electrical
  109 : Subsystem
  109 Y PQ : Subsystem  mask(Single Phase ZIP Load){Vnom=1.0*2401.78, fnom=60, Pnom=40e3*a, Qnom=20e3*a, LoadType=constant P, Vlim=0.7}
      mask prompts: Vnom "Nominal Voltage Vn (Vrms)"; fnom "Nominal Frequency fn (Hz)"; Pnom "Nominal Active power (W)"; Qnom "Nominal Reactive power (VAR)"; LoadType "Load Type"; Vlim "Minimum voltage (pu)"
      mask help:
      | Notes:
      | Single Phase ZIP load model which gets converted to constant Z type if the voltage becomes lower than the Minimum Voltage.
      mask TypeOptions LoadType: Constant Z | constant I | constant P
      mask DialogControl ParameterTabVar0 Prompt: Parameters
      mask DialogControl ParameterTabVar1 Prompt: Type
      mask Display:
      | color('red');
      | A=[-210,-180,-170,-160,-147,-140,-130,-120,-110,-80,-50,-49,-45,-39,-33,-26,-21,-18,-17,-19,-22,-22,-26,-27,-25,-22,-16,-9,-3,2,6,6,4,1,1,-3,-4,-2,2,7,14,20,26,29,30,28,24,24,21,20,21,25,31,37,44,49,50,50,80];
      | B=[-41.5,-41.5,-63,-20,-63,-20,-63,-20,-41.5,-41.5,-41.5,-34,-26,-21,-20,-22,-28,-37,-47,-57,-63,-63,-54,-44,-34,-26,-21,-20,-22,-28,-37,-47,-57,-63,-63,-54,-44,-34,-26,-21,-20,-22,-28,-37,-47,-57,-63,-63,-54,-44,-34,-26,-21,-20,-22,-28,-37,-41.50,-41.5];
      | plot(A,B);
      | color('black');
      | port_label('LConn', 1, '+')
  109-110 9 : powerlib/Elements/Distributed Parameters Line  Phases=1  Frequency=60  Resistance=R_9(1,1)  Inductance=L_9(1,1)  Capacitance=C_9(1,1)  Length=300*ft2km  x1=[3458.20413088381;376.991118430775;-0.010022883480317]  x2=[3458.20347144976;376.991118430775;-0.0100232996228292]  x3=[6.3186934920062;376.991118430775;-0.0108894511282481]  x4=[6.346355283731;376.991118430775;-0.00930042046484595]  x5=3.71926621942778e-07  V1=[2.049e+04;377;-2.115]  V2=[2.048e+04;377;-2.115]  I1=[33.62;377;-2.106]  I2=[35.2;377;-2.126]  nHarmo=1  Measurements=None
      settings: SourceProductName=Simscape Electrical
  11 : Subsystem
  11 Y Z : Subsystem  mask(Single Phase ZIP Load){Vnom=1.0*2401.78, fnom=60, Pnom=40e3*a, Qnom=20e3*a, LoadType=Constant Z, Vlim=0.7}
      mask prompts: Vnom "Nominal Voltage Vn (Vrms)"; fnom "Nominal Frequency fn (Hz)"; Pnom "Nominal Active power (W)"; Qnom "Nominal Reactive power (VAR)"; LoadType "Load Type"; Vlim "Minimum voltage (pu)"
      mask help:
      | Notes:
      | Single Phase ZIP load model which gets converted to constant Z type if the voltage becomes lower than the Minimum Voltage.
      mask TypeOptions LoadType: Constant Z | constant I | constant P
      mask DialogControl ParameterTabVar0 Prompt: Parameters
      mask DialogControl ParameterTabVar1 Prompt: Type
      mask Display:
      | color('red');
      | A=[-210,-180,-170,-160,-147,-140,-130,-120,-110,-80,-50,-49,-45,-39,-33,-26,-21,-18,-17,-19,-22,-22,-26,-27,-25,-22,-16,-9,-3,2,6,6,4,1,1,-3,-4,-2,2,7,14,20,26,29,30,28,24,24,21,20,21,25,31,37,44,49,50,50,80];
      | B=[-41.5,-41.5,-63,-20,-63,-20,-63,-20,-41.5,-41.5,-41.5,-34,-26,-21,-20,-22,-28,-37,-47,-57,-63,-63,-54,-44,-34,-26,-21,-20,-22,-28,-37,-47,-57,-63,-63,-54,-44,-34,-26,-21,-20,-22,-28,-37,-47,-57,-63,-63,-54,-44,-34,-26,-21,-20,-22,-28,-37,-41.50,-41.5];
      | plot(A,B);
      | color('black');
      | port_label('LConn', 1, '+')
  110 : Subsystem
  110-111 9 : powerlib/Elements/Distributed Parameters Line  Phases=1  Frequency=60  Resistance=R_9(1,1)  Inductance=L_9(1,1)  Capacitance=C_9(1,1)  Length=575*ft2km  x1=[3458.20347144975;376.991118430775;-0.0101518282365779]  x2=[3458.20309574629;376.991118430775;-0.0101520106023384]  x3=[6.32846214976806;376.991118430775;-0.0104207344047612]  x4=[6.33537672297077;376.991118430775;-0.0101520106171577]  x5=7.12859358723659e-07  V1=[2.049e+04;377;-2.115]  V2=[2.048e+04;377;-2.115]  I1=[33.62;377;-2.106]  I2=[35.2;377;-2.126]  nHarmo=1  Measurements=None
      settings: SourceProductName=Simscape Electrical
  110-112 9 : powerlib/Elements/Distributed Parameters Line  Phases=1  Frequency=60  Resistance=R_9(1,1)  Inductance=L_9(1,1)  Capacitance=C_9(1,1)  Length=125*ft2km  x1=[3458.20347144976;376.991118430775;-0.00994150868680736]  x2=[3458.20323114703;376.991118430775;-0.00994162896768818]  x3=[6.32253130803728;376.991118430775;-0.0103979546469382]  x4=[6.34327932903304;376.991118430775;-0.00954500317788115]  x5=1.54969425809491e-07  V1=[2.049e+04;377;-2.115]  V2=[2.048e+04;377;-2.115]  I1=[33.62;377;-2.106]  I2=[35.2;377;-2.126]  nHarmo=1  Measurements=None
      settings: SourceProductName=Simscape Electrical
  111 : Subsystem
  111 Y PQ : Subsystem  mask(Single Phase ZIP Load){Vnom=1.0*2401.78, fnom=60, Pnom=20e3*a, Qnom=10e3*a, LoadType=constant P, Vlim=0.7}
      mask prompts: Vnom "Nominal Voltage Vn (Vrms)"; fnom "Nominal Frequency fn (Hz)"; Pnom "Nominal Active power (W)"; Qnom "Nominal Reactive power (VAR)"; LoadType "Load Type"; Vlim "Minimum voltage (pu)"
      mask help:
      | Notes:
      | Single Phase ZIP load model which gets converted to constant Z type if the voltage becomes lower than the Minimum Voltage.
      mask TypeOptions LoadType: Constant Z | constant I | constant P
      mask DialogControl ParameterTabVar0 Prompt: Parameters
      mask DialogControl ParameterTabVar1 Prompt: Type
      mask Display:
      | color('red');
      | A=[-210,-180,-170,-160,-147,-140,-130,-120,-110,-80,-50,-49,-45,-39,-33,-26,-21,-18,-17,-19,-22,-22,-26,-27,-25,-22,-16,-9,-3,2,6,6,4,1,1,-3,-4,-2,2,7,14,20,26,29,30,28,24,24,21,20,21,25,31,37,44,49,50,50,80];
      | B=[-41.5,-41.5,-63,-20,-63,-20,-63,-20,-41.5,-41.5,-41.5,-34,-26,-21,-20,-22,-28,-37,-47,-57,-63,-63,-54,-44,-34,-26,-21,-20,-22,-28,-37,-47,-57,-63,-63,-54,-44,-34,-26,-21,-20,-22,-28,-37,-47,-57,-63,-63,-54,-44,-34,-26,-21,-20,-22,-28,-37,-41.50,-41.5];
      | plot(A,B);
      | color('black');
      | port_label('LConn', 1, '+')
  112 : Subsystem
  112 Y I : Subsystem  mask(Single Phase ZIP Load){Vnom=1.0*2401.78, fnom=60, Pnom=20e3*a, Qnom=10e3*a, LoadType=constant I, Vlim=0.7}
      mask prompts: Vnom "Nominal Voltage Vn (Vrms)"; fnom "Nominal Frequency fn (Hz)"; Pnom "Nominal Active power (W)"; Qnom "Nominal Reactive power (VAR)"; LoadType "Load Type"; Vlim "Minimum voltage (pu)"
      mask help:
      | Notes:
      | Single Phase ZIP load model which gets converted to constant Z type if the voltage becomes lower than the Minimum Voltage.
      mask TypeOptions LoadType: Constant Z | constant I | constant P
      mask DialogControl ParameterTabVar0 Prompt: Parameters
      mask DialogControl ParameterTabVar1 Prompt: Type
      mask Display:
      | color('red');
      | A=[-210,-180,-170,-160,-147,-140,-130,-120,-110,-80,-50,-49,-45,-39,-33,-26,-21,-18,-17,-19,-22,-22,-26,-27,-25,-22,-16,-9,-3,2,6,6,4,1,1,-3,-4,-2,2,7,14,20,26,29,30,28,24,24,21,20,21,25,31,37,44,49,50,50,80];
      | B=[-41.5,-41.5,-63,-20,-63,-20,-63,-20,-41.5,-41.5,-41.5,-34,-26,-21,-20,-22,-28,-37,-47,-57,-63,-63,-54,-44,-34,-26,-21,-20,-22,-28,-37,-47,-57,-63,-63,-54,-44,-34,-26,-21,-20,-22,-28,-37,-47,-57,-63,-63,-54,-44,-34,-26,-21,-20,-22,-28,-37,-41.50,-41.5];
      | plot(A,B);
      | color('black');
      | port_label('LConn', 1, '+')
  112-113 9 : powerlib/Elements/Distributed Parameters Line  Phases=1  Frequency=60  Resistance=R_9(1,1)  Inductance=L_9(1,1)  Capacitance=C_9(1,1)  Length=525*ft2km  x1=[3458.20323114703;376.991118430775;-0.0101285796785954]  x2=[3458.20255003728;376.991118430775;-0.0101289141083211]  x3=[6.32511362656628;376.991118430775;-0.0105263078461446]  x4=[6.33894308837021;376.991118430775;-0.00997717326433322]  x5=6.50871588399862e-07  V1=[2.049e+04;377;-2.115]  V2=[2.048e+04;377;-2.115]  I1=[33.62;377;-2.106]  I2=[35.2;377;-2.126]  nHarmo=1  Measurements=None
      settings: SourceProductName=Simscape Electrical
  113 : Subsystem
  113 Y Z : Subsystem  mask(Single Phase ZIP Load){Vnom=1.0*2401.78, fnom=60, Pnom=40e3*a, Qnom=20e3*a, LoadType=Constant Z, Vlim=0.7}
      mask prompts: Vnom "Nominal Voltage Vn (Vrms)"; fnom "Nominal Frequency fn (Hz)"; Pnom "Nominal Active power (W)"; Qnom "Nominal Reactive power (VAR)"; LoadType "Load Type"; Vlim "Minimum voltage (pu)"
      mask help:
      | Notes:
      | Single Phase ZIP load model which gets converted to constant Z type if the voltage becomes lower than the Minimum Voltage.
      mask TypeOptions LoadType: Constant Z | constant I | constant P
      mask DialogControl ParameterTabVar0 Prompt: Parameters
      mask DialogControl ParameterTabVar1 Prompt: Type
      mask Display:
      | color('red');
      | A=[-210,-180,-170,-160,-147,-140,-130,-120,-110,-80,-50,-49,-45,-39,-33,-26,-21,-18,-17,-19,-22,-22,-26,-27,-25,-22,-16,-9,-3,2,6,6,4,1,1,-3,-4,-2,2,7,14,20,26,29,30,28,24,24,21,20,21,25,31,37,44,49,50,50,80];
      | B=[-41.5,-41.5,-63,-20,-63,-20,-63,-20,-41.5,-41.5,-41.5,-34,-26,-21,-20,-22,-28,-37,-47,-57,-63,-63,-54,-44,-34,-26,-21,-20,-22,-28,-37,-47,-57,-63,-63,-54,-44,-34,-26,-21,-20,-22,-28,-37,-47,-57,-63,-63,-54,-44,-34,-26,-21,-20,-22,-28,-37,-41.50,-41.5];
      | plot(A,B);
      | color('black');
      | port_label('LConn', 1, '+')
  113-114 9 : powerlib/Elements/Distributed Parameters Line  Phases=1  Frequency=60  Resistance=R_9(1,1)  Inductance=L_9(1,1)  Capacitance=C_9(1,1)  Length=325*ft2km  x1=[3458.20255003728;376.991118430775;-0.0100354387528675]  x2=[3458.20230699455;376.991118430775;-0.010035533075526]  x3=[6.32900747291422;376.991118430775;-0.0101874248425073]  x4=[6.33592284160667;376.991118430775;-0.0100355330648287]  x5=4.02920507104677e-07  V1=[2.049e+04;377;-2.115]  V2=[2.048e+04;377;-2.115]  I1=[33.62;377;-2.106]  I2=[35.2;377;-2.126]  nHarmo=1  Measurements=None
      settings: SourceProductName=Simscape Electrical
  114 : Subsystem
  114 Y PQ : Subsystem  mask(Single Phase ZIP Load){Vnom=1.0*2401.78, fnom=60, Pnom=20e3*a, Qnom=10e3*a, LoadType=constant P, Vlim=0.7}
      mask prompts: Vnom "Nominal Voltage Vn (Vrms)"; fnom "Nominal Frequency fn (Hz)"; Pnom "Nominal Active power (W)"; Qnom "Nominal Reactive power (VAR)"; LoadType "Load Type"; Vlim "Minimum voltage (pu)"
      mask help:
      | Notes:
      | Single Phase ZIP load model which gets converted to constant Z type if the voltage becomes lower than the Minimum Voltage.
      mask TypeOptions LoadType: Constant Z | constant I | constant P
      mask DialogControl ParameterTabVar0 Prompt: Parameters
      mask DialogControl ParameterTabVar1 Prompt: Type
      mask Display:
      | color('red');
      | A=[-210,-180,-170,-160,-147,-140,-130,-120,-110,-80,-50,-49,-45,-39,-33,-26,-21,-18,-17,-19,-22,-22,-26,-27,-25,-22,-16,-9,-3,2,6,6,4,1,1,-3,-4,-2,2,7,14,20,26,29,30,28,24,24,21,20,21,25,31,37,44,49,50,50,80];
      | B=[-41.5,-41.5,-63,-20,-63,-20,-63,-20,-41.5,-41.5,-41.5,-34,-26,-21,-20,-22,-28,-37,-47,-57,-63,-63,-54,-44,-34,-26,-21,-20,-22,-28,-37,-47,-57,-63,-63,-54,-44,-34,-26,-21,-20,-22,-28,-37,-47,-57,-63,-63,-54,-44,-34,-26,-21,-20,-22,-28,-37,-41.50,-41.5];
      | plot(A,B);
      | color('black');
      | port_label('LConn', 1, '+')
  12 : Subsystem
  12 Y PQ : Subsystem  mask(Single Phase ZIP Load){Vnom=1.0*2401.78, fnom=60, Pnom=20e3*a, Qnom=10e3*a, LoadType=constant P, Vlim=0.7}
      mask prompts: Vnom "Nominal Voltage Vn (Vrms)"; fnom "Nominal Frequency fn (Hz)"; Pnom "Nominal Active power (W)"; Qnom "Nominal Reactive power (VAR)"; LoadType "Load Type"; Vlim "Minimum voltage (pu)"
      mask help:
      | Notes:
      | Single Phase ZIP load model which gets converted to constant Z type if the voltage becomes lower than the Minimum Voltage.
      mask TypeOptions LoadType: Constant Z | constant I | constant P
      mask DialogControl ParameterTabVar0 Prompt: Parameters
      mask DialogControl ParameterTabVar1 Prompt: Type
      mask Display:
      | color('red');
      | A=[-210,-180,-170,-160,-147,-140,-130,-120,-110,-80,-50,-49,-45,-39,-33,-26,-21,-18,-17,-19,-22,-22,-26,-27,-25,-22,-16,-9,-3,2,6,6,4,1,1,-3,-4,-2,2,7,14,20,26,29,30,28,24,24,21,20,21,25,31,37,44,49,50,50,80];
      | B=[-41.5,-41.5,-63,-20,-63,-20,-63,-20,-41.5,-41.5,-41.5,-34,-26,-21,-20,-22,-28,-37,-47,-57,-63,-63,-54,-44,-34,-26,-21,-20,-22,-28,-37,-47,-57,-63,-63,-54,-44,-34,-26,-21,-20,-22,-28,-37,-47,-57,-63,-63,-54,-44,-34,-26,-21,-20,-22,-28,-37,-41.50,-41.5];
      | plot(A,B);
      | color('black');
      | port_label('LConn', 1, '+')
  13 : powerlib/Measurements/Three-Phase V-I Measurement  VoltageMeasurement=phase-to-ground  SetLabelV=on  LabelV=V13  Vpu=off  VpuLL=off  CurrentMeasurement=no  SetLabelI=on  LabelI=I800  Ipu=off  Pbase=100e6  Vbase=24900  OutputType=Complex  PhasorSimulation=on  PSBequivalent=0
      settings: SourceProductName=Simscape Electrical
  13-152 : powerlib/Elements/Three-Phase Breaker  InitialState=closed  SwitchA=off  SwitchB=off  SwitchC=off  SwitchTimes=50  External=off  BreakerResistance=1e-6  SnubberResistance=1e6  SnubberCapacitance=inf  Measurements=None
      settings: SourceProductName=Simscape Electrical
  13-18 2 : powerlib/Elements/Distributed Parameters Line  Phases=3  Frequency=60  Resistance=R_2  Inductance=L_2  Capacitance=C_2  Length=825*ft2km  x1=[440.131582208599 4187.39406017362 4181.67769888773;376.991118430775 376.991118430775 376.991118430775;-2.49762834364949 -0.311685786037419 -1.88123859919816]  x2=[440.133540310574 4187.39532633519 4181.67893678406;376.991118430775 376.991118430775 376.991118430775;-2.49762056943124 -0.311687421615739 -1.88124002918139]  x3=[0.59066017492404 15.5747250034349 12.2829655382627;376.991118430775 376.991118430775 376.991118430775;-2.50069575918239 -0.314712468279924 -1.88380807177098]  x4=[0.566240345195593 15.6834527728283 12.3665124175991;376.991118430775 376.991118430775 376.991118430775;-2.49481918908358 -0.309004238545016 -1.87900905538041]  x5=1.03467372757201e-06  V1=ones(3,3)  V2=ones(3,3)  I1=ones(3,3)  I2=ones(3,3)  nHarmo=1  Measurements=None
      settings: SourceProductName=Simscape Electrical
  13-34 11 : powerlib/Elements/Distributed Parameters Line  Phases=1  Frequency=60  Resistance=R_11(3,3)  Inductance=L_11(3,3)  Capacitance=C_11(3,3)  Length=150*ft2km  x1=[3419.45355486823;376.991118430775;2.09165303164435]  x2=[3419.45326743883;376.991118430775;2.09165288517473]  x3=[6.25150541068841;376.991118430775;2.09118035480385]  x4=[6.27227379125216;376.991118430775;2.09205400550066]  x5=1.85963310971389e-07  V1=[2.049e+04;377;-2.115]  V2=[2.048e+04;377;-2.115]  I1=[33.62;377;-2.106]  I2=[35.2;377;-2.126]  nHarmo=1  Measurements=None
      settings: SourceProductName=Simscape Electrical
  135 : powerlib/Measurements/Three-Phase V-I Measurement  VoltageMeasurement=phase-to-ground  SetLabelV=on  LabelV=V135  Vpu=off  VpuLL=off  CurrentMeasurement=no  SetLabelI=on  LabelI=I800  Ipu=off  Pbase=100e6  Vbase=24900  OutputType=Complex  PhasorSimulation=on  PSBequivalent=0
      settings: SourceProductName=Simscape Electrical
  135-35 4 : powerlib/Elements/Distributed Parameters Line  Phases=3  Frequency=60  Resistance=R_4  Inductance=L_4  Capacitance=C_4  Length=375*ft2km  x1=[438.08385821254 4184.3182267772 4184.78559496153;376.991118430775 376.991118430775 376.991118430775;0.395103775173951 -0.220017293918831 -1.78946421067745]  x2=[438.083110038637 4184.31874511349 4184.78547638917;376.991118430775 376.991118430775 376.991118430775;0.395102202451055 -0.220017779517276 -1.789464564299]  x3=[0.569483695069589 12.3027088331924 15.5903795183729;376.991118430775 376.991118430775 376.991118430775;0.400303984525805 -0.222022062001551 -1.79040892838536]  x4=[0.582115262360279 12.36372695859 15.6504882844907;376.991118430775 376.991118430775 376.991118430775;0.389839472045612 -0.218169009579599 -1.78867029899729]  x5=4.70306239805458e-07  V1=ones(3,3)  V2=ones(3,3)  I1=ones(3,3)  I2=ones(3,3)  nHarmo=1  Measurements=None
      settings: SourceProductName=Simscape Electrical
  14 : Subsystem
  14-10 9 : powerlib/Elements/Distributed Parameters Line  Phases=1  Frequency=60  Resistance=R_9(1,1)  Inductance=L_9(1,1)  Capacitance=C_9(1,1)  Length=250*ft2km  x1=[3412.46787917345;376.991118430775;-0.00328611688771187]  x2=[3412.46807064526;376.991118430775;-0.00328604635189753]  x3=[6.25229291403514;376.991118430775;-0.00328611689502728]  x4=[6.24546876484087;376.991118430775;-0.00340295770377142]  x5=3.09938851618982e-07  V1=[2.049e+04;377;-2.115]  V2=[2.048e+04;377;-2.115]  I1=[33.62;377;-2.106]  I2=[35.2;377;-2.126]  nHarmo=1  Measurements=None
      settings: SourceProductName=Simscape Electrical
  14-11 9 : powerlib/Elements/Distributed Parameters Line  Phases=1  Frequency=60  Resistance=R_9(1,1)  Inductance=L_9(1,1)  Capacitance=C_9(1,1)  Length=250*ft2km  x1=[3412.46807064526;376.991118430775;-0.00328604635189753]  x2=[3412.46787917345;376.991118430775;-0.0032861168877119]  x3=[6.24546876484454;376.991118430775;-0.00340295770551689]  x4=[6.25229291402784;376.991118430775;-0.00328611689386731]  x5=3.09938851618982e-07  V1=[2.049e+04;377;-2.115]  V2=[2.048e+04;377;-2.115]  I1=[33.62;377;-2.106]  I2=[35.2;377;-2.126]  nHarmo=1  Measurements=None
      settings: SourceProductName=Simscape Electrical
  149 : powerlib/Measurements/Three-Phase V-I Measurement  VoltageMeasurement=phase-to-ground  SetLabelV=on  LabelV=V149  Vpu=off  VpuLL=off  CurrentMeasurement=no  SetLabelI=on  LabelI=I800  Ipu=off  Pbase=100e6  Vbase=24900  OutputType=Complex  PhasorSimulation=on  PSBequivalent=0
      settings: SourceProductName=Simscape Electrical
  149-1 1 : powerlib/Elements/Distributed Parameters Line  Phases=3  Frequency=60  Resistance=R_1  Inductance=L_1  Capacitance=C_1  Length=400*ft2km  x1=[436.4522737793 4159.57354594326 4157.02975526765;376.991118430775 376.991118430775 376.991118430775;1.69154828464408 -2.40210672387619 2.31025168170426]  x2=[436.800297543745 4167.29457653455 4166.80094747361;376.991118430775 376.991118430775 376.991118430775;1.69101871639727 -2.40316801567855 2.30919177551073]  x3=[2.63872692974907 185.681714359137 185.599075217066;376.991118430775 376.991118430775 376.991118430775;0.130064949448095 2.37798283077441 0.792822551456475]  x4=[2.86733668227892 186.160933404381 185.896806021162;376.991118430775 376.991118430775 376.991118430775;2.85985146549455 -0.93095994031386 -2.48094012389847]  x5=5.01659989125821e-07  V1=ones(3,3)  V2=ones(3,3)  I1=ones(3,3)  I2=ones(3,3)  nHarmo=1  Measurements=None
      settings: SourceProductName=Simscape Electrical
  15 : Subsystem
  15-16 11 : powerlib/Elements/Distributed Parameters Line  Phases=1  Frequency=60  Resistance=R_11(3,3)  Inductance=L_11(3,3)  Capacitance=C_11(3,3)  Length=375*ft2km  x1=[3419.45315316264;376.991118430775;2.09154765765879]  x2=[3419.45288287366;376.991118430775;2.09154754680489]  x3=[6.25798232301171;376.991118430775;2.09137228808747]  x4=[6.26482004658177;376.991118430775;2.09154754681353]  x5=4.64908277428473e-07  V1=[2.049e+04;377;-2.115]  V2=[2.048e+04;377;-2.115]  I1=[33.62;377;-2.106]  I2=[35.2;377;-2.126]  nHarmo=1  Measurements=None
      settings: SourceProductName=Simscape Electrical
  15-17 11 : powerlib/Elements/Distributed Parameters Line  Phases=1  Frequency=60  Resistance=R_11(3,3)  Inductance=L_11(3,3)  Capacitance=C_11(3,3)  Length=350*ft2km  x1=[3419.45315316264;376.991118430775;2.09155934207822]  x2=[3419.45289762502;376.991118430775;2.09155923955728]  x3=[6.25803641581959;376.991118430775;2.09139566428849]  x4=[6.26487421823574;376.991118430775;2.09155923956058]  x5=4.33914392266575e-07  V1=[2.049e+04;377;-2.115]  V2=[2.048e+04;377;-2.115]  I1=[33.62;377;-2.106]  I2=[35.2;377;-2.126]  nHarmo=1  Measurements=None
      settings: SourceProductName=Simscape Electrical
  150 : powerlib/Measurements/Three-Phase V-I Measurement  VoltageMeasurement=phase-to-ground  SetLabelV=on  LabelV=V150  Vpu=off  VpuLL=off  CurrentMeasurement=yes  SetLabelI=on  LabelI=I150  Ipu=off  Pbase=100e6  Vbase=24900  OutputType=Complex  PhasorSimulation=on  PSBequivalent=0
      settings: SourceProductName=Simscape Electrical
  150-1 : powerlib/Elements/Three-Phase Breaker  InitialState=closed  SwitchA=off  SwitchB=off  SwitchC=off  SwitchTimes="[1/60  5/60]"  External=off  BreakerResistance=1e-6  SnubberResistance=1e6  SnubberCapacitance=inf  Measurements=None
      settings: SourceProductName=Simscape Electrical
  151 : powerlib/Measurements/Three-Phase V-I Measurement  VoltageMeasurement=phase-to-ground  SetLabelV=on  LabelV=V151  Vpu=off  VpuLL=off  CurrentMeasurement=no  SetLabelI=on  LabelI=I65  Ipu=off  Pbase=100e6  Vbase=24900  OutputType=Complex  PhasorSimulation=on  PSBequivalent=0
      settings: SourceProductName=Simscape Electrical
  151-1 : powerlib/Elements/Three-Phase Breaker  InitialState=open  SwitchA=off  SwitchB=off  SwitchC=off  SwitchTimes="[1/60  5/60]"  External=off  BreakerResistance=0.01  SnubberResistance=1e6  SnubberCapacitance=inf  Measurements=None
      settings: SourceProductName=Simscape Electrical
  152 : powerlib/Measurements/Three-Phase V-I Measurement  VoltageMeasurement=phase-to-ground  SetLabelV=on  LabelV=V152  Vpu=off  VpuLL=off  CurrentMeasurement=no  SetLabelI=on  LabelI=I65  Ipu=off  Pbase=100e6  Vbase=24900  OutputType=Complex  PhasorSimulation=on  PSBequivalent=0
      settings: SourceProductName=Simscape Electrical
  152-52 1 : powerlib/Elements/Distributed Parameters Line  Phases=3  Frequency=60  Resistance=R_1  Inductance=L_1  Capacitance=C_1  Length=400*ft2km  x1=[437.497229772424 4182.75074086414 4186.35705747284;376.991118430775 376.991118430775 376.991118430775;1.68996347549705 -2.40527867949513 2.30708716247487]  x2=[437.848330578358 4190.48566193662 4196.1402512421;376.991118430775 376.991118430775 376.991118430775;1.68943875243625 -2.40632740215243 2.30604326075919]  x3=[2.65362058543645 185.704886375293 185.581593325858;376.991118430775 376.991118430775 376.991118430775;0.135265481454682 2.37878806562029 0.793663001396626]  x4=[2.87487037285329 186.077458739336 185.79460657557;376.991118430775 376.991118430775 376.991118430775;2.86519116496016 -0.931124169281442 -2.48108038589907]  x5=5.01659989125821e-07  V1=ones(3,3)  V2=ones(3,3)  I1=ones(3,3)  I2=ones(3,3)  nHarmo=1  Measurements=None
      settings: SourceProductName=Simscape Electrical
  16 : Subsystem
  16 Y PQ : Subsystem  mask(Single Phase ZIP Load){Vnom=1.0*2401.78, fnom=60, Pnom=40e3*a, Qnom=20e3*a, LoadType=constant P, Vlim=0.7}
      mask prompts: Vnom "Nominal Voltage Vn (Vrms)"; fnom "Nominal Frequency fn (Hz)"; Pnom "Nominal Active power (W)"; Qnom "Nominal Reactive power (VAR)"; LoadType "Load Type"; Vlim "Minimum voltage (pu)"
      mask help:
      | Notes:
      | Single Phase ZIP load model which gets converted to constant Z type if the voltage becomes lower than the Minimum Voltage.
      mask TypeOptions LoadType: Constant Z | constant I | constant P
      mask DialogControl ParameterTabVar0 Prompt: Parameters
      mask DialogControl ParameterTabVar1 Prompt: Type
      mask Display:
      | color('red');
      | A=[-210,-180,-170,-160,-147,-140,-130,-120,-110,-80,-50,-49,-45,-39,-33,-26,-21,-18,-17,-19,-22,-22,-26,-27,-25,-22,-16,-9,-3,2,6,6,4,1,1,-3,-4,-2,2,7,14,20,26,29,30,28,24,24,21,20,21,25,31,37,44,49,50,50,80];
      | B=[-41.5,-41.5,-63,-20,-63,-20,-63,-20,-41.5,-41.5,-41.5,-34,-26,-21,-20,-22,-28,-37,-47,-57,-63,-63,-54,-44,-34,-26,-21,-20,-22,-28,-37,-47,-57,-63,-63,-54,-44,-34,-26,-21,-20,-22,-28,-37,-47,-57,-63,-63,-54,-44,-34,-26,-21,-20,-22,-28,-37,-41.50,-41.5];
      | plot(A,B);
      | color('black');
      | port_label('LConn', 1, '+')
  160 : powerlib/Measurements/Three-Phase V-I Measurement  VoltageMeasurement=phase-to-ground  SetLabelV=on  LabelV=V160  Vpu=off  VpuLL=off  CurrentMeasurement=no  SetLabelI=on  LabelI=I65  Ipu=off  Pbase=100e6  Vbase=24900  OutputType=Complex  PhasorSimulation=on  PSBequivalent=0
      settings: SourceProductName=Simscape Electrical
  160 67 6 : powerlib/Elements/Distributed Parameters Line  Phases=3  Frequency=60  Resistance=R_3  Inductance=L_3  Capacitance=C_3  Length=350*ft2km  x1=[443.077137701126 4223.67526683416 4225.38226587948;376.991118430775 376.991118430775 376.991118430775;-0.41656278823488 0.206950603849322 1.77982310987574]  x2=[443.372743388461 4232.25893017917 4232.16211805871;376.991118430775 376.991118430775 376.991118430775;-0.417011941237458 0.206054323278974 1.77892412057173]  x3=[2.56893002782851 185.758803048561 185.576550732056;376.991118430775 376.991118430775 376.991118430775;-1.97523930834198 -1.30106582313234 0.286945252737006]  x4=[2.80757484849076 185.854281411043 185.787974450509;376.991118430775 376.991118430775 376.991118430775;0.738461807029519 1.70628874132578 -3.02486720329101]  x5=4.38952490485094e-07  V1=ones(3,3)  V2=ones(3,3)  I1=ones(3,3)  I2=ones(3,3)  nHarmo=1  Measurements=None
      settings: SourceProductName=Simscape Electrical
  17 : Subsystem
  17 Y PQ : Subsystem  mask(Single Phase ZIP Load){Vnom=1.0*2401.78, fnom=60, Pnom=20e3*a, Qnom=10e3*a, LoadType=constant P, Vlim=0.7}
      mask prompts: Vnom "Nominal Voltage Vn (Vrms)"; fnom "Nominal Frequency fn (Hz)"; Pnom "Nominal Active power (W)"; Qnom "Nominal Reactive power (VAR)"; LoadType "Load Type"; Vlim "Minimum voltage (pu)"
      mask help:
      | Notes:
      | Single Phase ZIP load model which gets converted to constant Z type if the voltage becomes lower than the Minimum Voltage.
      mask TypeOptions LoadType: Constant Z | constant I | constant P
      mask DialogControl ParameterTabVar0 Prompt: Parameters
      mask DialogControl ParameterTabVar1 Prompt: Type
      mask Display:
      | color('red');
      | A=[-210,-180,-170,-160,-147,-140,-130,-120,-110,-80,-50,-49,-45,-39,-33,-26,-21,-18,-17,-19,-22,-22,-26,-27,-25,-22,-16,-9,-3,2,6,6,4,1,1,-3,-4,-2,2,7,14,20,26,29,30,28,24,24,21,20,21,25,31,37,44,49,50,50,80];
      | B=[-41.5,-41.5,-63,-20,-63,-20,-63,-20,-41.5,-41.5,-41.5,-34,-26,-21,-20,-22,-28,-37,-47,-57,-63,-63,-54,-44,-34,-26,-21,-20,-22,-28,-37,-47,-57,-63,-63,-54,-44,-34,-26,-21,-20,-22,-28,-37,-47,-57,-63,-63,-54,-44,-34,-26,-21,-20,-22,-28,-37,-41.50,-41.5];
      | plot(A,B);
      | color('black');
      | port_label('LConn', 1, '+')
  18 : powerlib/Measurements/Three-Phase V-I Measurement  VoltageMeasurement=phase-to-ground  SetLabelV=on  LabelV=V18  Vpu=off  VpuLL=off  CurrentMeasurement=no  SetLabelI=on  LabelI=I800  Ipu=off  Pbase=100e6  Vbase=24900  OutputType=Complex  PhasorSimulation=on  PSBequivalent=0
      settings: SourceProductName=Simscape Electrical
  18-135 : powerlib/Elements/Three-Phase Breaker  InitialState=closed  SwitchA=off  SwitchB=off  SwitchC=off  SwitchTimes=10  External=off  BreakerResistance=1e-6  SnubberResistance=1e6  SnubberCapacitance=inf  Measurements=None
      settings: SourceProductName=Simscape Electrical
  18-19 9 : powerlib/Elements/Distributed Parameters Line  Phases=1  Frequency=60  Resistance=R_9(1,1)  Inductance=L_9(1,1)  Capacitance=C_9(1,1)  Length=250*ft2km  x1=[3417.75992520928;376.991118430775;-0.00433701163595883]  x2=[3417.759576844;376.991118430775;-0.00433716330548609]  x3=[6.25172435892621;376.991118430775;-0.00460256166227999]  x4=[6.26541807251049;376.991118430775;-0.00418891337035581]  x5=3.09938851618982e-07  V1=[2.049e+04;377;-2.115]  V2=[2.048e+04;377;-2.115]  I1=[33.62;377;-2.106]  I2=[35.2;377;-2.126]  nHarmo=1  Measurements=None
      settings: SourceProductName=Simscape Electrical
  18-21 2 : powerlib/Elements/Distributed Parameters Line  Phases=3  Frequency=60  Resistance=R_2  Inductance=L_2  Capacitance=C_2  Length=300*ft2km  x1=[440.133540310574 4187.39532633519 4181.67893678406;376.991118430775 376.991118430775 376.991118430775;-2.49737234764575 -0.311481475708237 -1.88103497905633]  x2=[440.133207998065 4187.39541674067 4181.67936488531;376.991118430775 376.991118430775 376.991118430775;-2.49737082667424 -0.31148167341146 -1.88103512985221]  x3=[0.582790840538662 15.6114518200797 12.3161737205416;376.991118430775 376.991118430775 376.991118430775;-2.4892130921232 -0.312392766701396 -1.88230036900827]  x4=[0.574232974301385 15.6492794973206 12.3349120264936;376.991118430775 376.991118430775 376.991118430775;-2.50579457208529 -0.310690128016207 -1.87988874607368]  x5=3.76244991844366e-07  V1=ones(3,3)  V2=ones(3,3)  I1=ones(3,3)  I2=ones(3,3)  nHarmo=1  Measurements=None
      settings: SourceProductName=Simscape Electrical
  19 : Subsystem
  19 Y PQ : Subsystem  mask(Single Phase ZIP Load){Vnom=1.0*2401.78, fnom=60, Pnom=40e3*a, Qnom=20e3*a, LoadType=constant P, Vlim=0.7}
      mask prompts: Vnom "Nominal Voltage Vn (Vrms)"; fnom "Nominal Frequency fn (Hz)"; Pnom "Nominal Active power (W)"; Qnom "Nominal Reactive power (VAR)"; LoadType "Load Type"; Vlim "Minimum voltage (pu)"
      mask help:
      | Notes:
      | Single Phase ZIP load model which gets converted to constant Z type if the voltage becomes lower than the Minimum Voltage.
      mask TypeOptions LoadType: Constant Z | constant I | constant P
      mask DialogControl ParameterTabVar0 Prompt: Parameters
      mask DialogControl ParameterTabVar1 Prompt: Type
      mask Display:
      | color('red');
      | A=[-210,-180,-170,-160,-147,-140,-130,-120,-110,-80,-50,-49,-45,-39,-33,-26,-21,-18,-17,-19,-22,-22,-26,-27,-25,-22,-16,-9,-3,2,6,6,4,1,1,-3,-4,-2,2,7,14,20,26,29,30,28,24,24,21,20,21,25,31,37,44,49,50,50,80];
      | B=[-41.5,-41.5,-63,-20,-63,-20,-63,-20,-41.5,-41.5,-41.5,-34,-26,-21,-20,-22,-28,-37,-47,-57,-63,-63,-54,-44,-34,-26,-21,-20,-22,-28,-37,-47,-57,-63,-63,-54,-44,-34,-26,-21,-20,-22,-28,-37,-47,-57,-63,-63,-54,-44,-34,-26,-21,-20,-22,-28,-37,-41.50,-41.5];
      | plot(A,B);
      | color('black');
      | port_label('LConn', 1, '+')
  19-20 9 : powerlib/Elements/Distributed Parameters Line  Phases=1  Frequency=60  Resistance=R_9(1,1)  Inductance=L_9(1,1)  Capacitance=C_9(1,1)  Length=325*ft2km  x1=[3417.759576844;376.991118430775;-0.00437221656378118]  x2=[3417.75933665005;376.991118430775;-0.00437231088642371]  x3=[6.25499106112965;376.991118430775;-0.00452420889896637]  x4=[6.26182547759843;376.991118430775;-0.00437230463608164]  x5=4.02920507104677e-07  V1=[2.049e+04;377;-2.115]  V2=[2.048e+04;377;-2.115]  I1=[33.62;377;-2.106]  I2=[35.2;377;-2.126]  nHarmo=1  Measurements=None
      settings: SourceProductName=Simscape Electrical
  197 : powerlib/Measurements/Three-Phase V-I Measurement  VoltageMeasurement=phase-to-ground  SetLabelV=on  LabelV=V197  Vpu=off  VpuLL=off  CurrentMeasurement=no  SetLabelI=on  LabelI=I65  Ipu=off  Pbase=100e6  Vbase=24900  OutputType=Complex  PhasorSimulation=on  PSBequivalent=0
      settings: SourceProductName=Simscape Electrical
  197-101 3 : powerlib/Elements/Distributed Parameters Line  Phases=3  Frequency=60  Resistance=R_3  Inductance=L_3  Capacitance=C_3  Length=250*ft2km  x1=[443.373227080419 4232.2593632027 4232.16270174298;376.991118430775 376.991118430775 376.991118430775;-0.416965831815374 0.206093045513335 1.77896306468544]  x2=[443.373660115841 4232.25950788553 4232.16299468928;376.991118430775 376.991118430775 376.991118430775;-0.416966855382457 0.206092867530335 1.77896294086887]  x3=[0.580101891122803 12.4572135777982 15.7870308679579;376.991118430775 376.991118430775 376.991118430775;-0.427181556050575 0.205080078013259 1.77783812806618]  x4=[0.585467222055824 12.4921970599795 15.8081724856609;376.991118430775 376.991118430775 376.991118430775;-0.406962409081875 0.207005491301578 1.7799883678684]  x5=3.13537493203638e-07  V1=ones(3,3)  V2=ones(3,3)  I1=ones(3,3)  I2=ones(3,3)  nHarmo=1  Measurements=None
      settings: SourceProductName=Simscape Electrical
  2 : Subsystem
  2 Y PQ : Subsystem  mask(Single Phase ZIP Load){Vnom=1.0*2401.78, fnom=60, Pnom=20e3*a, Qnom=10e3*a, LoadType=constant P, Vlim=0.7}
      mask prompts: Vnom "Nominal Voltage Vn (Vrms)"; fnom "Nominal Frequency fn (Hz)"; Pnom "Nominal Active power (W)"; Qnom "Nominal Reactive power (VAR)"; LoadType "Load Type"; Vlim "Minimum voltage (pu)"
      mask help:
      | Notes:
      | Single Phase ZIP load model which gets converted to constant Z type if the voltage becomes lower than the Minimum Voltage.
      mask TypeOptions LoadType: Constant Z | constant I | constant P
      mask DialogControl ParameterTabVar0 Prompt: Parameters
      mask DialogControl ParameterTabVar1 Prompt: Type
      mask Display:
      | color('red');
      | A=[-210,-180,-170,-160,-147,-140,-130,-120,-110,-80,-50,-49,-45,-39,-33,-26,-21,-18,-17,-19,-22,-22,-26,-27,-25,-22,-16,-9,-3,2,6,6,4,1,1,-3,-4,-2,2,7,14,20,26,29,30,28,24,24,21,20,21,25,31,37,44,49,50,50,80];
      | B=[-41.5,-41.5,-63,-20,-63,-20,-63,-20,-41.5,-41.5,-41.5,-34,-26,-21,-20,-22,-28,-37,-47,-57,-63,-63,-54,-44,-34,-26,-21,-20,-22,-28,-37,-47,-57,-63,-63,-54,-44,-34,-26,-21,-20,-22,-28,-37,-47,-57,-63,-63,-54,-44,-34,-26,-21,-20,-22,-28,-37,-41.50,-41.5];
      | plot(A,B);
      | color('black');
      | port_label('LConn', 1, '+')
  20 : Subsystem
  20 Y I : Subsystem  mask(Single Phase ZIP Load){Vnom=1.0*2401.78, fnom=60, Pnom=40e3*a, Qnom=20e3*a, LoadType=constant I, Vlim=0.7}
      mask prompts: Vnom "Nominal Voltage Vn (Vrms)"; fnom "Nominal Frequency fn (Hz)"; Pnom "Nominal Active power (W)"; Qnom "Nominal Reactive power (VAR)"; LoadType "Load Type"; Vlim "Minimum voltage (pu)"
      mask help:
      | Notes:
      | Single Phase ZIP load model which gets converted to constant Z type if the voltage becomes lower than the Minimum Voltage.
      mask TypeOptions LoadType: Constant Z | constant I | constant P
      mask DialogControl ParameterTabVar0 Prompt: Parameters
      mask DialogControl ParameterTabVar1 Prompt: Type
      mask Display:
      | color('red');
      | A=[-210,-180,-170,-160,-147,-140,-130,-120,-110,-80,-50,-49,-45,-39,-33,-26,-21,-18,-17,-19,-22,-22,-26,-27,-25,-22,-16,-9,-3,2,6,6,4,1,1,-3,-4,-2,2,7,14,20,26,29,30,28,24,24,21,20,21,25,31,37,44,49,50,50,80];
      | B=[-41.5,-41.5,-63,-20,-63,-20,-63,-20,-41.5,-41.5,-41.5,-34,-26,-21,-20,-22,-28,-37,-47,-57,-63,-63,-54,-44,-34,-26,-21,-20,-22,-28,-37,-47,-57,-63,-63,-54,-44,-34,-26,-21,-20,-22,-28,-37,-47,-57,-63,-63,-54,-44,-34,-26,-21,-20,-22,-28,-37,-41.50,-41.5];
      | plot(A,B);
      | color('black');
      | port_label('LConn', 1, '+')
  21 : powerlib/Measurements/Three-Phase V-I Measurement  VoltageMeasurement=phase-to-ground  SetLabelV=on  LabelV=V21  Vpu=off  VpuLL=off  CurrentMeasurement=no  SetLabelI=on  LabelI=I800  Ipu=off  Pbase=100e6  Vbase=24900  OutputType=Complex  PhasorSimulation=on  PSBequivalent=0
      settings: SourceProductName=Simscape Electrical
  21-22 10 : powerlib/Elements/Distributed Parameters Line  Phases=1  Frequency=60  Resistance=R_10(2,2)  Inductance=L_10(2,2)  Capacitance=C_10(2,2)  Length=525*ft2km  x1=[3416.97134491207;376.991118430775;-2.09725675295332]  x2=[3416.97099439355;376.991118430775;-2.09725691646934]  x3=[6.25311152262213;376.991118430775;-2.09750086523843]  x4=[6.25995284690995;376.991118430775;-2.09725832444523]  x5=6.50871588399862e-07  V1=[2.049e+04;377;-2.115]  V2=[2.048e+04;377;-2.115]  I1=[33.62;377;-2.106]  I2=[35.2;377;-2.126]  nHarmo=1  Measurements=None
      settings: SourceProductName=Simscape Electrical
  21-23 2 : powerlib/Elements/Distributed Parameters Line  Phases=3  Frequency=60  Resistance=R_2  Inductance=L_2  Capacitance=C_2  Length=250*ft2km  x1=[440.133207998065 4187.39541674067 4181.67936488531;376.991118430775 376.991118430775 376.991118430775;-2.49734718650419 -0.311462059515508 -1.88101560126887]  x2=[440.132822706747 4187.39543265634 4181.6796988423;376.991118430775 376.991118430775 376.991118430775;-2.49734547511547 -0.311462217886438 -1.88101569914038]  x3=[0.584266871403802 15.6113998227784 12.3189449489567;376.991118430775 376.991118430775 376.991118430775;-2.48613517954281 -0.312224924169043 -1.88211956163414]  x4=[0.57279942137908 15.6495822956098 12.3322965560309;376.991118430775 376.991118430775 376.991118430775;-2.50890132474281 -0.310799165478228 -1.88001052502927]  x5=3.13537493203638e-07  V1=ones(3,3)  V2=ones(3,3)  I1=ones(3,3)  I2=ones(3,3)  nHarmo=1  Measurements=None
      settings: SourceProductName=Simscape Electrical
  22 : Subsystem
  22 Y Z : Subsystem  mask(Single Phase ZIP Load){Vnom=1.0*2401.78, fnom=60, Pnom=40e3*a, Qnom=20e3*a, LoadType=Constant Z, Vlim=0.7}
      mask prompts: Vnom "Nominal Voltage Vn (Vrms)"; fnom "Nominal Frequency fn (Hz)"; Pnom "Nominal Active power (W)"; Qnom "Nominal Reactive power (VAR)"; LoadType "Load Type"; Vlim "Minimum voltage (pu)"
      mask help:
      | Notes:
      | Single Phase ZIP load model which gets converted to constant Z type if the voltage becomes lower than the Minimum Voltage.
      mask TypeOptions LoadType: Constant Z | constant I | constant P
      mask DialogControl ParameterTabVar0 Prompt: Parameters
      mask DialogControl ParameterTabVar1 Prompt: Type
      mask Display:
      | color('red');
      | A=[-210,-180,-170,-160,-147,-140,-130,-120,-110,-80,-50,-49,-45,-39,-33,-26,-21,-18,-17,-19,-22,-22,-26,-27,-25,-22,-16,-9,-3,2,6,6,4,1,1,-3,-4,-2,2,7,14,20,26,29,30,28,24,24,21,20,21,25,31,37,44,49,50,50,80];
      | B=[-41.5,-41.5,-63,-20,-63,-20,-63,-20,-41.5,-41.5,-41.5,-34,-26,-21,-20,-22,-28,-37,-47,-57,-63,-63,-54,-44,-34,-26,-21,-20,-22,-28,-37,-47,-57,-63,-63,-54,-44,-34,-26,-21,-20,-22,-28,-37,-47,-57,-63,-63,-54,-44,-34,-26,-21,-20,-22,-28,-37,-41.50,-41.5];
      | plot(A,B);
      | color('black');
      | port_label('LConn', 1, '+')
  23 : powerlib/Measurements/Three-Phase V-I Measurement  VoltageMeasurement=phase-to-ground  SetLabelV=on  LabelV=V23  Vpu=off  VpuLL=off  CurrentMeasurement=no  SetLabelI=on  LabelI=I800  Ipu=off  Pbase=100e6  Vbase=24900  OutputType=Complex  PhasorSimulation=on  PSBequivalent=0
      settings: SourceProductName=Simscape Electrical
  23-24 11 : powerlib/Elements/Distributed Parameters Line  Phases=1  Frequency=60  Resistance=R_11(3,3)  Inductance=L_11(3,3)  Capacitance=C_11(3,3)  Length=550*ft2km  x1=[3419.45212250801;376.991118430775;2.09146422799282]  x2=[3419.45176327328;376.991118430775;2.09146405545843]  x3=[6.25761144705111;376.991118430775;2.09120711725866]  x4=[6.26442937607704;376.991118430775;2.09146395283017]  x5=6.8186547356176e-07  V1=[2.049e+04;377;-2.115]  V2=[2.048e+04;377;-2.115]  I1=[33.62;377;-2.106]  I2=[35.2;377;-2.126]  nHarmo=1  Measurements=None
      settings: SourceProductName=Simscape Electrical
  23-25 2 : powerlib/Elements/Distributed Parameters Line  Phases=3  Frequency=60  Resistance=R_2  Inductance=L_2  Capacitance=C_2  Length=275*ft2km  x1=[440.132822706747 4187.39543265634 4181.6796988423;376.991118430775 376.991118430775 376.991118430775;-2.4973572952005 -0.311472024834414 -1.88102546343205]  x2=[440.132631881892 4187.39545606589 4181.6799506362;376.991118430775 376.991118430775 376.991118430775;-2.49735544436818 -0.311472180793873 -1.88102555192074]  x3=[0.58493709248048 15.6134489656746 12.3195870817988;376.991118430775 376.991118430775 376.991118430775;-2.48971591860705 -0.312178079513607 -1.88185258084818]  x4=[0.572084493955744 15.6474050920201 12.3315709444921;376.991118430775 376.991118430775 376.991118430775;-2.50529996002757 -0.310875419125002 -1.88030659453618]  x5=3.44891242524002e-07  V1=ones(3,3)  V2=ones(3,3)  I1=ones(3,3)  I2=ones(3,3)  nHarmo=1  Measurements=None
      settings: SourceProductName=Simscape Electrical
  24 : Subsystem
  24 Y PQ : Subsystem  mask(Single Phase ZIP Load){Vnom=1.0*2401.78, fnom=60, Pnom=40e3*a, Qnom=20e3*a, LoadType=constant P, Vlim=0.7}
      mask prompts: Vnom "Nominal Voltage Vn (Vrms)"; fnom "Nominal Frequency fn (Hz)"; Pnom "Nominal Active power (W)"; Qnom "Nominal Reactive power (VAR)"; LoadType "Load Type"; Vlim "Minimum voltage (pu)"
      mask help:
      | Notes:
      | Single Phase ZIP load model which gets converted to constant Z type if the voltage becomes lower than the Minimum Voltage.
      mask TypeOptions LoadType: Constant Z | constant I | constant P
      mask DialogControl ParameterTabVar0 Prompt: Parameters
      mask DialogControl ParameterTabVar1 Prompt: Type
      mask Display:
      | color('red');
      | A=[-210,-180,-170,-160,-147,-140,-130,-120,-110,-80,-50,-49,-45,-39,-33,-26,-21,-18,-17,-19,-22,-22,-26,-27,-25,-22,-16,-9,-3,2,6,6,4,1,1,-3,-4,-2,2,7,14,20,26,29,30,28,24,24,21,20,21,25,31,37,44,49,50,50,80];
      | B=[-41.5,-41.5,-63,-20,-63,-20,-63,-20,-41.5,-41.5,-41.5,-34,-26,-21,-20,-22,-28,-37,-47,-57,-63,-63,-54,-44,-34,-26,-21,-20,-22,-28,-37,-47,-57,-63,-63,-54,-44,-34,-26,-21,-20,-22,-28,-37,-47,-57,-63,-63,-54,-44,-34,-26,-21,-20,-22,-28,-37,-41.50,-41.5];
      | plot(A,B);
      | color('black');
      | port_label('LConn', 1, '+')
  25 : powerlib/Measurements/Three-Phase V-I Measurement  VoltageMeasurement=phase-to-ground  SetLabelV=on  LabelV=V25  Vpu=off  VpuLL=off  CurrentMeasurement=no  SetLabelI=on  LabelI=I800  Ipu=off  Pbase=100e6  Vbase=24900  OutputType=Complex  PhasorSimulation=on  PSBequivalent=0
      settings: SourceProductName=Simscape Electrical
  25-26 1 : powerlib/Elements/Distributed Parameters Line  Phases=2  Frequency=60  Resistance=R_7([1 3],[1 3])  Inductance=L_7([1 3],[1 3])  Capacitance=C_7([1 3],[1 3])  Length=350*ft2km  x1=[4188.37252663888 2413.60261690792;376.991118430775 376.991118430775;-0.526786058282874 1.03415249509051]  x2=[4188.37252658063 2413.60286235825;376.991118430775 376.991118430775;-0.526786140698572 1.03415228536988]  x3=[12.5789314242924 4.04191971699812;376.991118430775 376.991118430775;-0.527078609645416 1.03307291097648]  x4=[12.5915879077714 4.04901213258006;376.991118430775 376.991118430775;-0.526630562593711 1.03506837260057]  x5=4.29041749824869e-07  V1=ones(3,3)  V2=ones(3,3)  I1=ones(3,3)  I2=ones(3,3)  nHarmo=1  Measurements=None
      settings: SourceProductName=Simscape Electrical
  25-28 2 : powerlib/Elements/Distributed Parameters Line  Phases=3  Frequency=60  Resistance=R_2  Inductance=L_2  Capacitance=C_2  Length=200*ft2km  x1=[440.132631881892 4187.39545606589 4181.6799506362;376.991118430775 376.991118430775 376.991118430775;-2.49731998411311 -0.311442759949944 -1.88099625904573]  x2=[440.132774825681 4187.39550823897 4181.68003778237;376.991118430775 376.991118430775 376.991118430775;-2.49731947734574 -0.3114428109147 -1.88099628320047]  x3=[0.581856769462903 15.6238827862569 12.3237007350559;376.991118430775 376.991118430775 376.991118430775;-2.49846710509597 -0.31187872443767 -1.88137285104822]  x4=[0.575142685473116 15.6373480695961 12.327688923124;376.991118430775 376.991118430775 376.991118430775;-2.49625407563007 -0.311085644470139 -1.88069791539081]  x5=2.50829994562911e-07  V1=ones(3,3)  V2=ones(3,3)  I1=ones(3,3)  I2=ones(3,3)  nHarmo=1  Measurements=None
      settings: SourceProductName=Simscape Electrical
  250 : powerlib/Measurements/Three-Phase V-I Measurement  VoltageMeasurement=phase-to-ground  SetLabelV=on  LabelV=V250  Vpu=off  VpuLL=off  CurrentMeasurement=no  SetLabelI=on  LabelI=I800  Ipu=off  Pbase=100e6  Vbase=24900  OutputType=Complex  PhasorSimulation=on  PSBequivalent=0
      settings: SourceProductName=Simscape Electrical
  250-251 : powerlib/Elements/Three-Phase Breaker  InitialState=open  SwitchA=on  SwitchB=on  SwitchC=on  SwitchTimes="[1/60  5/60]"  External=off  BreakerResistance=0.01  SnubberResistance=1e6  SnubberCapacitance=inf  Measurements=None
      settings: SourceProductName=Simscape Electrical
  26 : Subsystem
  26-27 7 : powerlib/Elements/Distributed Parameters Line  Phases=2  Frequency=60  Resistance=R_7([1 3],[1 3])  Inductance=L_7([1 3],[1 3])  Capacitance=C_7([1 3],[1 3])  Length=275*ft2km  x1=[4188.37252658063 2413.60286235825;376.991118430775 376.991118430775;-0.526756838009192 1.03418694499755]  x2=[4188.37260048963 2413.60269630272;376.991118430775 376.991118430775;-0.526756861934673 1.03418689570482]  x3=[12.5838136539378 4.04339238299749;376.991118430775 376.991118430775;-0.527030417182466 1.03444471678517]  x4=[12.5869524186769 4.04762451614688;376.991118430775 376.991118430775;-0.526590782063122 1.03380237290706]  x5=3.37104232005254e-07  V1=ones(3,3)  V2=ones(3,3)  I1=ones(3,3)  I2=ones(3,3)  nHarmo=1  Measurements=None
      settings: SourceProductName=Simscape Electrical
  26-31 1 : powerlib/Elements/Distributed Parameters Line  Phases=1  Frequency=60  Resistance=R_11(3,3)  Inductance=L_11(3,3)  Capacitance=C_11(3,3)  Length=225*ft2km  x1=[3419.45175793319;376.991118430775;2.09161576408061]  x2=[3419.45143988901;376.991118430775;2.09161562923782]  x3=[6.25488522665443;376.991118430775;2.09137011648174]  x4=[6.26856161416105;376.991118430775;2.09175569326122]  x5=2.78944966457084e-07  V1=[2.049e+04;377;-2.115]  V2=[2.048e+04;377;-2.115]  I1=[33.62;377;-2.106]  I2=[35.2;377;-2.126]  nHarmo=1  Measurements=None
      settings: SourceProductName=Simscape Electrical
  27 : Subsystem
  27-33 1 : powerlib/Elements/Distributed Parameters Line  Phases=1  Frequency=60  Resistance=R_9(1,1)  Inductance=L_9(1,1)  Capacitance=C_9(1,1)  Length=500*ft2km  x1=[3417.76147072947;376.991118430775;-0.00445464905924852]  x2=[3417.76113385333;376.991118430775;-0.0044548035983601]  x3=[6.2546160415356;376.991118430775;-0.00468847939558361]  x4=[6.26144999523548;376.991118430775;-0.00445480270866001]  x5=6.19877703237964e-07  V1=[2.049e+04;377;-2.115]  V2=[2.048e+04;377;-2.115]  I1=[33.62;377;-2.106]  I2=[35.2;377;-2.126]  nHarmo=1  Measurements=None
      settings: SourceProductName=Simscape Electrical
  28 : powerlib/Measurements/Three-Phase V-I Measurement  VoltageMeasurement=phase-to-ground  SetLabelV=on  LabelV=V28  Vpu=off  VpuLL=off  CurrentMeasurement=no  SetLabelI=on  LabelI=I800  Ipu=off  Pbase=100e6  Vbase=24900  OutputType=Complex  PhasorSimulation=on  PSBequivalent=0
      settings: SourceProductName=Simscape Electrical
  28 Y I : Subsystem  mask(Single Phase ZIP Load){Vnom=1.0*2401.78, fnom=60, Pnom=40e3*a, Qnom=20e3*a, LoadType=constant I, Vlim=0.7}
      mask prompts: Vnom "Nominal Voltage Vn (Vrms)"; fnom "Nominal Frequency fn (Hz)"; Pnom "Nominal Active power (W)"; Qnom "Nominal Reactive power (VAR)"; LoadType "Load Type"; Vlim "Minimum voltage (pu)"
      mask help:
      | Notes:
      | Single Phase ZIP load model which gets converted to constant Z type if the voltage becomes lower than the Minimum Voltage.
      mask TypeOptions LoadType: Constant Z | constant I | constant P
      mask DialogControl ParameterTabVar0 Prompt: Parameters
      mask DialogControl ParameterTabVar1 Prompt: Type
      mask Display:
      | color('red');
      | A=[-210,-180,-170,-160,-147,-140,-130,-120,-110,-80,-50,-49,-45,-39,-33,-26,-21,-18,-17,-19,-22,-22,-26,-27,-25,-22,-16,-9,-3,2,6,6,4,1,1,-3,-4,-2,2,7,14,20,26,29,30,28,24,24,21,20,21,25,31,37,44,49,50,50,80];
      | B=[-41.5,-41.5,-63,-20,-63,-20,-63,-20,-41.5,-41.5,-41.5,-34,-26,-21,-20,-22,-28,-37,-47,-57,-63,-63,-54,-44,-34,-26,-21,-20,-22,-28,-37,-47,-57,-63,-63,-54,-44,-34,-26,-21,-20,-22,-28,-37,-47,-57,-63,-63,-54,-44,-34,-26,-21,-20,-22,-28,-37,-41.50,-41.5];
      | plot(A,B);
      | color('black');
      | port_label('LConn', 1, '+')
  28-29 2 : powerlib/Elements/Distributed Parameters Line  Phases=3  Frequency=60  Resistance=R_2  Inductance=L_2  Capacitance=C_2  Length=300*ft2km  x1=[440.132774825681 4187.39550823897 4181.68003778237;376.991118430775 376.991118430775 376.991118430775;-2.49736675768583 -0.311482038706606 -1.88103534036715]  x2=[440.132787243053 4187.39555777282 4181.68016432889;376.991118430775 376.991118430775 376.991118430775;-2.49736625627647 -0.311482085351865 -1.88103537271204]  x3=[0.580292773821334 15.6262770616396 12.3238481305123;376.991118430775 376.991118430775 376.991118430775;-2.49639046678108 -0.311785694388071 -1.88141213103237]  x4=[0.576690357524223 15.6344450693053 12.3272265445439;376.991118430775 376.991118430775 376.991118430775;-2.49849093025887 -0.311296242844164 -1.88077584224845]  x5=3.76244991844366e-07  V1=ones(3,3)  V2=ones(3,3)  I1=ones(3,3)  I2=ones(3,3)  nHarmo=1  Measurements=None
      settings: SourceProductName=Simscape Electrical
  29 : powerlib/Measurements/Three-Phase V-I Measurement  VoltageMeasurement=phase-to-ground  SetLabelV=on  LabelV=V29  Vpu=off  VpuLL=off  CurrentMeasurement=no  SetLabelI=on  LabelI=I800  Ipu=off  Pbase=100e6  Vbase=24900  OutputType=Complex  PhasorSimulation=on  PSBequivalent=0
      settings: SourceProductName=Simscape Electrical
  29 Y Z : Subsystem  mask(Single Phase ZIP Load){Vnom=1.0*2401.78, fnom=60, Pnom=40e3*a, Qnom=20e3*a, LoadType=Constant Z, Vlim=0.7}
      mask prompts: Vnom "Nominal Voltage Vn (Vrms)"; fnom "Nominal Frequency fn (Hz)"; Pnom "Nominal Active power (W)"; Qnom "Nominal Reactive power (VAR)"; LoadType "Load Type"; Vlim "Minimum voltage (pu)"
      mask help:
      | Notes:
      | Single Phase ZIP load model which gets converted to constant Z type if the voltage becomes lower than the Minimum Voltage.
      mask TypeOptions LoadType: Constant Z | constant I | constant P
      mask DialogControl ParameterTabVar0 Prompt: Parameters
      mask DialogControl ParameterTabVar1 Prompt: Type
      mask Display:
      | color('red');
      | A=[-210,-180,-170,-160,-147,-140,-130,-120,-110,-80,-50,-49,-45,-39,-33,-26,-21,-18,-17,-19,-22,-22,-26,-27,-25,-22,-16,-9,-3,2,6,6,4,1,1,-3,-4,-2,2,7,14,20,26,29,30,28,24,24,21,20,21,25,31,37,44,49,50,50,80];
      | B=[-41.5,-41.5,-63,-20,-63,-20,-63,-20,-41.5,-41.5,-41.5,-34,-26,-21,-20,-22,-28,-37,-47,-57,-63,-63,-54,-44,-34,-26,-21,-20,-22,-28,-37,-47,-57,-63,-63,-54,-44,-34,-26,-21,-20,-22,-28,-37,-47,-57,-63,-63,-54,-44,-34,-26,-21,-20,-22,-28,-37,-41.50,-41.5];
      | plot(A,B);
      | color('black');
      | port_label('LConn', 1, '+')
  29-30 2 : powerlib/Elements/Distributed Parameters Line  Phases=3  Frequency=60  Resistance=R_2  Inductance=L_2  Capacitance=C_2  Length=350*ft2km  x1=[440.132787243053 4187.39555777282 4181.68016432889;376.991118430775 376.991118430775 376.991118430775;-2.49738989644651 -0.311501699247818 -1.88105490129538]  x2=[440.132563483977 4187.39556513339 4181.68029035326;376.991118430775 376.991118430775 376.991118430775;-2.49738961097523 -0.31150171666907 -1.88105493274633]  x3=[0.578735486369586 15.6287983308506 12.3240743435445;376.991118430775 376.991118430775 376.991118430775;-2.4942315196831 -0.311633855865988 -1.88139282692251]  x4=[0.578244582262644 15.6316693558954 12.3268430005812;376.991118430775 376.991118430775 376.991118430775;-2.50071622311613 -0.311506871587565 -1.88085376978699]  x5=4.38952490485094e-07  V1=ones(3,3)  V2=ones(3,3)  I1=ones(3,3)  I2=ones(3,3)  nHarmo=1  Measurements=None
      settings: SourceProductName=Simscape Electrical
  3 : Subsystem
  3-4 11 : powerlib/Elements/Distributed Parameters Line  Phases=1  Frequency=60  Resistance=R_11(3,3)  Inductance=L_11(3,3)  Capacitance=C_11(3,3)  Length=200*ft2km  x1=[3404.23180903077;376.991118430775;2.09340652513952]  x2=[3404.23165250024;376.991118430775;2.09340646978798]  x3=[6.23050249642384;376.991118430775;2.09331300263732]  x4=[6.23731044125337;376.991118430775;2.09340646374663]  x5=2.47951081295186e-07  V1=[2.049e+04;377;-2.115]  V2=[2.048e+04;377;-2.115]  I1=[33.62;377;-2.106]  I2=[35.2;377;-2.126]  nHarmo=1  Measurements=None
      settings: SourceProductName=Simscape Electrical
  3-5 11 : powerlib/Elements/Distributed Parameters Line  Phases=1  Frequency=60  Resistance=R_11(3,3)  Inductance=L_11(3,3)  Capacitance=C_11(3,3)  Length=325*ft2km  x1=[3404.23180903077;376.991118430775;2.09334810304236]  x2=[3404.23135167358;376.991118430775;2.09334790826926]  x3=[6.22682940727421;376.991118430775;2.09307906150782]  x4=[6.24044435928389;376.991118430775;2.09346462560421]  x5=4.02920507104677e-07  V1=[2.049e+04;377;-2.115]  V2=[2.048e+04;377;-2.115]  I1=[33.62;377;-2.106]  I2=[35.2;377;-2.126]  nHarmo=1  Measurements=None
      settings: SourceProductName=Simscape Electrical
  "30 " : powerlib/Measurements/Three-Phase V-I Measurement  VoltageMeasurement=phase-to-ground  SetLabelV=on  LabelV=V30  Vpu=off  VpuLL=off  CurrentMeasurement=no  SetLabelI=on  LabelI=I800  Ipu=off  Pbase=100e6  Vbase=24900  OutputType=Complex  PhasorSimulation=on  PSBequivalent=0
      settings: SourceProductName=Simscape Electrical
  30 Y PQ : Subsystem  mask(Single Phase ZIP Load){Vnom=1.0*2401.78, fnom=60, Pnom=40e3*a, Qnom=20e3*a, LoadType=constant P, Vlim=0.7}
      mask prompts: Vnom "Nominal Voltage Vn (Vrms)"; fnom "Nominal Frequency fn (Hz)"; Pnom "Nominal Active power (W)"; Qnom "Nominal Reactive power (VAR)"; LoadType "Load Type"; Vlim "Minimum voltage (pu)"
      mask help:
      | Notes:
      | Single Phase ZIP load model which gets converted to constant Z type if the voltage becomes lower than the Minimum Voltage.
      mask TypeOptions LoadType: Constant Z | constant I | constant P
      mask DialogControl ParameterTabVar0 Prompt: Parameters
      mask DialogControl ParameterTabVar1 Prompt: Type
      mask Display:
      | color('red');
      | A=[-210,-180,-170,-160,-147,-140,-130,-120,-110,-80,-50,-49,-45,-39,-33,-26,-21,-18,-17,-19,-22,-22,-26,-27,-25,-22,-16,-9,-3,2,6,6,4,1,1,-3,-4,-2,2,7,14,20,26,29,30,28,24,24,21,20,21,25,31,37,44,49,50,50,80];
      | B=[-41.5,-41.5,-63,-20,-63,-20,-63,-20,-41.5,-41.5,-41.5,-34,-26,-21,-20,-22,-28,-37,-47,-57,-63,-63,-54,-44,-34,-26,-21,-20,-22,-28,-37,-47,-57,-63,-63,-54,-44,-34,-26,-21,-20,-22,-28,-37,-47,-57,-63,-63,-54,-44,-34,-26,-21,-20,-22,-28,-37,-41.50,-41.5];
      | plot(A,B);
      | color('black');
      | port_label('LConn', 1, '+')
  30-250 2 : powerlib/Elements/Distributed Parameters Line  Phases=3  Frequency=60  Resistance=R_2  Inductance=L_2  Capacitance=C_2  Length=200*ft2km  x1=[440.132563483977 4187.39556513339 4181.68029035326;376.991118430775 376.991118430775 376.991118430775;-2.49731869046509 -0.311442874981212 -1.88099634699631]  x2=[440.132565451755 4187.39557802069 4181.68030311125;376.991118430775 376.991118430775 376.991118430775;-2.4973186922587 -0.311442876679826 -1.88099634832923]  x3=[0.578499191488414 15.6306145447808 12.3256950284106;376.991118430775 376.991118430775 376.991118430775;-2.49741325214174 -0.311521331423965 -1.88107446199327]  x4=[0.578499191349536 15.6306145449045 12.3256950283063;376.991118430775 376.991118430775 376.991118430775;-2.49731869214489 -0.3114428766739 -1.88099634833141]  x5=2.50829994562911e-07  V1=ones(3,3)  V2=ones(3,3)  I1=ones(3,3)  I2=ones(3,3)  nHarmo=1  Measurements=None
      settings: SourceProductName=Simscape Electrical
  300 : powerlib/Measurements/Three-Phase V-I Measurement  VoltageMeasurement=phase-to-ground  SetLabelV=on  LabelV=V300  Vpu=off  VpuLL=off  CurrentMeasurement=no  SetLabelI=on  LabelI=I65  Ipu=off  Pbase=100e6  Vbase=24900  OutputType=Complex  PhasorSimulation=on  PSBequivalent=0
      settings: SourceProductName=Simscape Electrical
  300-1 : powerlib/Elements/Three-Phase Breaker  InitialState=open  SwitchA=off  SwitchB=off  SwitchC=off  SwitchTimes="[1/60  5/60]"  External=off  BreakerResistance=0.01  SnubberResistance=1e6  SnubberCapacitance=inf  Measurements=None
      settings: SourceProductName=Simscape Electrical
  31 : Subsystem
  31 Y PQ : Subsystem  mask(Single Phase ZIP Load){Vnom=1.0*2401.78, fnom=60, Pnom=20e3*a, Qnom=10e3*a, LoadType=constant P, Vlim=0.7}
      mask prompts: Vnom "Nominal Voltage Vn (Vrms)"; fnom "Nominal Frequency fn (Hz)"; Pnom "Nominal Active power (W)"; Qnom "Nominal Reactive power (VAR)"; LoadType "Load Type"; Vlim "Minimum voltage (pu)"
      mask help:
      | Notes:
      | Single Phase ZIP load model which gets converted to constant Z type if the voltage becomes lower than the Minimum Voltage.
      mask TypeOptions LoadType: Constant Z | constant I | constant P
      mask DialogControl ParameterTabVar0 Prompt: Parameters
      mask DialogControl ParameterTabVar1 Prompt: Type
      mask Display:
      | color('red');
      | A=[-210,-180,-170,-160,-147,-140,-130,-120,-110,-80,-50,-49,-45,-39,-33,-26,-21,-18,-17,-19,-22,-22,-26,-27,-25,-22,-16,-9,-3,2,6,6,4,1,1,-3,-4,-2,2,7,14,20,26,29,30,28,24,24,21,20,21,25,31,37,44,49,50,50,80];
      | B=[-41.5,-41.5,-63,-20,-63,-20,-63,-20,-41.5,-41.5,-41.5,-34,-26,-21,-20,-22,-28,-37,-47,-57,-63,-63,-54,-44,-34,-26,-21,-20,-22,-28,-37,-47,-57,-63,-63,-54,-44,-34,-26,-21,-20,-22,-28,-37,-47,-57,-63,-63,-54,-44,-34,-26,-21,-20,-22,-28,-37,-41.50,-41.5];
      | plot(A,B);
      | color('black');
      | port_label('LConn', 1, '+')
  31-32 1 : powerlib/Elements/Distributed Parameters Line  Phases=1  Frequency=60  Resistance=R_11(3,3)  Inductance=L_11(3,3)  Capacitance=C_11(3,3)  Length=300*ft2km  x1=[3419.45143988901;376.991118430775;2.09158057597953]  x2=[3419.45121525526;376.991118430775;2.09158048972087]  x3=[6.25814148172351;376.991118430775;2.09144028234044]  x4=[6.26497941496855;376.991118430775;2.09158048892343]  x5=3.71926621942778e-07  V1=[2.049e+04;377;-2.115]  V2=[2.048e+04;377;-2.115]  I1=[33.62;377;-2.106]  I2=[35.2;377;-2.126]  nHarmo=1  Measurements=None
      settings: SourceProductName=Simscape Electrical
  32 : Subsystem
  32 Y PQ : Subsystem  mask(Single Phase ZIP Load){Vnom=1.0*2401.78, fnom=60, Pnom=20e3*a, Qnom=10e3*a, LoadType=constant P, Vlim=0.7}
      mask prompts: Vnom "Nominal Voltage Vn (Vrms)"; fnom "Nominal Frequency fn (Hz)"; Pnom "Nominal Active power (W)"; Qnom "Nominal Reactive power (VAR)"; LoadType "Load Type"; Vlim "Minimum voltage (pu)"
      mask help:
      | Notes:
      | Single Phase ZIP load model which gets converted to constant Z type if the voltage becomes lower than the Minimum Voltage.
      mask TypeOptions LoadType: Constant Z | constant I | constant P
      mask DialogControl ParameterTabVar0 Prompt: Parameters
      mask DialogControl ParameterTabVar1 Prompt: Type
      mask Display:
      | color('red');
      | A=[-210,-180,-170,-160,-147,-140,-130,-120,-110,-80,-50,-49,-45,-39,-33,-26,-21,-18,-17,-19,-22,-22,-26,-27,-25,-22,-16,-9,-3,2,6,6,4,1,1,-3,-4,-2,2,7,14,20,26,29,30,28,24,24,21,20,21,25,31,37,44,49,50,50,80];
      | B=[-41.5,-41.5,-63,-20,-63,-20,-63,-20,-41.5,-41.5,-41.5,-34,-26,-21,-20,-22,-28,-37,-47,-57,-63,-63,-54,-44,-34,-26,-21,-20,-22,-28,-37,-47,-57,-63,-63,-54,-44,-34,-26,-21,-20,-22,-28,-37,-47,-57,-63,-63,-54,-44,-34,-26,-21,-20,-22,-28,-37,-41.50,-41.5];
      | plot(A,B);
      | color('black');
      | port_label('LConn', 1, '+')
  33 : Subsystem
  33 Y I : Subsystem  mask(Single Phase ZIP Load){Vnom=1.0*2401.78, fnom=60, Pnom=40e3*a, Qnom=20e3*a, LoadType=constant I, Vlim=0.7}
      mask prompts: Vnom "Nominal Voltage Vn (Vrms)"; fnom "Nominal Frequency fn (Hz)"; Pnom "Nominal Active power (W)"; Qnom "Nominal Reactive power (VAR)"; LoadType "Load Type"; Vlim "Minimum voltage (pu)"
      mask help:
      | Notes:
      | Single Phase ZIP load model which gets converted to constant Z type if the voltage becomes lower than the Minimum Voltage.
      mask TypeOptions LoadType: Constant Z | constant I | constant P
      mask DialogControl ParameterTabVar0 Prompt: Parameters
      mask DialogControl ParameterTabVar1 Prompt: Type
      mask Display:
      | color('red');
      | A=[-210,-180,-170,-160,-147,-140,-130,-120,-110,-80,-50,-49,-45,-39,-33,-26,-21,-18,-17,-19,-22,-22,-26,-27,-25,-22,-16,-9,-3,2,6,6,4,1,1,-3,-4,-2,2,7,14,20,26,29,30,28,24,24,21,20,21,25,31,37,44,49,50,50,80];
      | B=[-41.5,-41.5,-63,-20,-63,-20,-63,-20,-41.5,-41.5,-41.5,-34,-26,-21,-20,-22,-28,-37,-47,-57,-63,-63,-54,-44,-34,-26,-21,-20,-22,-28,-37,-47,-57,-63,-63,-54,-44,-34,-26,-21,-20,-22,-28,-37,-47,-57,-63,-63,-54,-44,-34,-26,-21,-20,-22,-28,-37,-41.50,-41.5];
      | plot(A,B);
      | color('black');
      | port_label('LConn', 1, '+')
  34 : Subsystem
  34 Y Z : Subsystem  mask(Single Phase ZIP Load){Vnom=1.0*2401.78, fnom=60, Pnom=40e3*a, Qnom=20e3*a, LoadType=Constant Z, Vlim=0.7}
      mask prompts: Vnom "Nominal Voltage Vn (Vrms)"; fnom "Nominal Frequency fn (Hz)"; Pnom "Nominal Active power (W)"; Qnom "Nominal Reactive power (VAR)"; LoadType "Load Type"; Vlim "Minimum voltage (pu)"
      mask help:
      | Notes:
      | Single Phase ZIP load model which gets converted to constant Z type if the voltage becomes lower than the Minimum Voltage.
      mask TypeOptions LoadType: Constant Z | constant I | constant P
      mask DialogControl ParameterTabVar0 Prompt: Parameters
      mask DialogControl ParameterTabVar1 Prompt: Type
      mask Display:
      | color('red');
      | A=[-210,-180,-170,-160,-147,-140,-130,-120,-110,-80,-50,-49,-45,-39,-33,-26,-21,-18,-17,-19,-22,-22,-26,-27,-25,-22,-16,-9,-3,2,6,6,4,1,1,-3,-4,-2,2,7,14,20,26,29,30,28,24,24,21,20,21,25,31,37,44,49,50,50,80];
      | B=[-41.5,-41.5,-63,-20,-63,-20,-63,-20,-41.5,-41.5,-41.5,-34,-26,-21,-20,-22,-28,-37,-47,-57,-63,-63,-54,-44,-34,-26,-21,-20,-22,-28,-37,-47,-57,-63,-63,-54,-44,-34,-26,-21,-20,-22,-28,-37,-47,-57,-63,-63,-54,-44,-34,-26,-21,-20,-22,-28,-37,-41.50,-41.5];
      | plot(A,B);
      | color('black');
      | port_label('LConn', 1, '+')
  34-15 11 : powerlib/Elements/Distributed Parameters Line  Phases=1  Frequency=60  Resistance=R_11(3,3)  Inductance=L_11(3,3)  Capacitance=C_11(3,3)  Length=100*ft2km  x1=[3419.45326743883;376.991118430775;2.09167625401359]  x2=[3419.45315316264;376.991118430775;2.09167618627254]  x3=[6.25515871394249;376.991118430775;2.0912902423682]  x4=[6.26883589429743;376.991118430775;2.09201466857193]  x5=1.23975540647593e-07  V1=[2.049e+04;377;-2.115]  V2=[2.048e+04;377;-2.115]  I1=[33.62;377;-2.106]  I2=[35.2;377;-2.126]  nHarmo=1  Measurements=None
      settings: SourceProductName=Simscape Electrical
  35 : powerlib/Measurements/Three-Phase V-I Measurement  VoltageMeasurement=phase-to-ground  SetLabelV=on  LabelV=V35  Vpu=off  VpuLL=off  CurrentMeasurement=no  SetLabelI=on  LabelI=I800  Ipu=off  Pbase=100e6  Vbase=24900  OutputType=Complex  PhasorSimulation=on  PSBequivalent=0
      settings: SourceProductName=Simscape Electrical
  35 D PQ : Subsystem  mask(Single Phase ZIP Load){Vnom=1.0*2401.78, fnom=60, Pnom=40e3*a, Qnom=20e3*a, LoadType=constant P, Vlim=0.7}
      mask prompts: Vnom "Nominal Voltage Vn (Vrms)"; fnom "Nominal Frequency fn (Hz)"; Pnom "Nominal Active power (W)"; Qnom "Nominal Reactive power (VAR)"; LoadType "Load Type"; Vlim "Minimum voltage (pu)"
      mask help:
      | Notes:
      | Single Phase ZIP load model which gets converted to constant Z type if the voltage becomes lower than the Minimum Voltage.
      mask TypeOptions LoadType: Constant Z | constant I | constant P
      mask DialogControl ParameterTabVar0 Prompt: Parameters
      mask DialogControl ParameterTabVar1 Prompt: Type
      mask Display:
      | color('red');
      | A=[-210,-180,-170,-160,-147,-140,-130,-120,-110,-80,-50,-49,-45,-39,-33,-26,-21,-18,-17,-19,-22,-22,-26,-27,-25,-22,-16,-9,-3,2,6,6,4,1,1,-3,-4,-2,2,7,14,20,26,29,30,28,24,24,21,20,21,25,31,37,44,49,50,50,80];
      | B=[-41.5,-41.5,-63,-20,-63,-20,-63,-20,-41.5,-41.5,-41.5,-34,-26,-21,-20,-22,-28,-37,-47,-57,-63,-63,-54,-44,-34,-26,-21,-20,-22,-28,-37,-47,-57,-63,-63,-54,-44,-34,-26,-21,-20,-22,-28,-37,-47,-57,-63,-63,-54,-44,-34,-26,-21,-20,-22,-28,-37,-41.50,-41.5];
      | plot(A,B);
      | color('black');
      | port_label('LConn', 1, '+')
  35-36 8 : powerlib/Elements/Distributed Parameters Line  Phases=2  Frequency=60  Resistance=R_8([1 2],[1 2])  Inductance=L_8([1 2],[1 2])  Capacitance=C_8([1 2],[1 2])  Length=650*ft2km  x1=[4183.04622340831 2419.32535746005;376.991118430775 376.991118430775;-2.62119196108045 -1.06054632998688]  x2=[4183.0463652379 2419.32495067506;376.991118430775 376.991118430775;-2.62119212114691 -1.06054661945104]  x3=[12.5627785812848 4.05074710361959;376.991118430775 376.991118430775;-2.62166493375716 -1.06056564240086]  x4=[12.5747481668403 4.05900867191404;376.991118430775 376.991118430775;-2.62097344156092 -1.06082743328286]  x5=7.96791821103328e-07  V1=ones(3,3)  V2=ones(3,3)  I1=ones(3,3)  I2=ones(3,3)  nHarmo=1  Measurements=None
      settings: SourceProductName=Simscape Electrical
  35-40 1 : powerlib/Elements/Distributed Parameters Line  Phases=3  Frequency=60  Resistance=R_1  Inductance=L_1  Capacitance=C_1  Length=250*ft2km  x1=[437.492294835355 4182.75149959783 4186.35928061438;376.991118430775 376.991118430775 376.991118430775;1.69003304524312 -2.40522172437837 2.30714383566038]  x2=[437.491775418153 4182.75150382427 4186.35948826417;376.991118430775 376.991118430775 376.991118430775;1.69003309652954 -2.40522189116136 2.30714358685808]  x3=[0.573265830916147 15.5928721012148 12.3153168998806;376.991118430775 376.991118430775 376.991118430775;1.69880287118542 -2.40599914568572 2.30573086685785]  x4=[0.576827627688831 15.6334411561128 12.3635217525362;376.991118430775 376.991118430775 376.991118430775;1.68119958645703 -2.40454443062356 2.30845359343131]  x5=3.13537493203638e-07  V1=ones(3,3)  V2=ones(3,3)  I1=ones(3,3)  I2=ones(3,3)  nHarmo=1  Measurements=None
      settings: SourceProductName=Simscape Electrical
  36 : Subsystem
  36-37 9 : powerlib/Elements/Distributed Parameters Line  Phases=1  Frequency=60  Resistance=R_9(1,1)  Inductance=L_9(1,1)  Capacitance=C_9(1,1)  Length=300*ft2km  x1=[3417.75967951611;376.991118430775;-0.00436112046618944]  x2=[3417.759454993;376.991118430775;-0.00436120672522672]  x3=[6.2550452787375;376.991118430775;-0.0045014149129533]  x4=[6.26187985233551;376.991118430775;-0.0043612067164933]  x5=3.71926621942778e-07  V1=[2.049e+04;377;-2.115]  V2=[2.048e+04;377;-2.115]  I1=[33.62;377;-2.106]  I2=[35.2;377;-2.126]  nHarmo=1  Measurements=None
      settings: SourceProductName=Simscape Electrical
  36-38 10 : powerlib/Elements/Distributed Parameters Line  Phases=1  Frequency=60  Resistance=R_10(2,2)  Inductance=L_10(2,2)  Capacitance=C_10(2,2)  Length=250*ft2km  x1=[3416.97152156773;376.991118430775;-2.09712893207352]  x2=[3416.97117543852;376.991118430775;-2.09712908391895]  x3=[6.25029434307812;376.991118430775;-2.09739797476315]  x4=[6.26396066611243;376.991118430775;-2.09697734814062]  x5=3.09938851618982e-07  V1=[2.049e+04;377;-2.115]  V2=[2.048e+04;377;-2.115]  I1=[33.62;377;-2.106]  I2=[35.2;377;-2.126]  nHarmo=1  Measurements=None
      settings: SourceProductName=Simscape Electrical
  37 : Subsystem
  37 Y Z : Subsystem  mask(Single Phase ZIP Load){Vnom=1.0*2401.78, fnom=60, Pnom=40e3*a, Qnom=20e3*a, LoadType=Constant Z, Vlim=0.7}
      mask prompts: Vnom "Nominal Voltage Vn (Vrms)"; fnom "Nominal Frequency fn (Hz)"; Pnom "Nominal Active power (W)"; Qnom "Nominal Reactive power (VAR)"; LoadType "Load Type"; Vlim "Minimum voltage (pu)"
      mask help:
      | Notes:
      | Single Phase ZIP load model which gets converted to constant Z type if the voltage becomes lower than the Minimum Voltage.
      mask TypeOptions LoadType: Constant Z | constant I | constant P
      mask DialogControl ParameterTabVar0 Prompt: Parameters
      mask DialogControl ParameterTabVar1 Prompt: Type
      mask Display:
      | color('red');
      | A=[-210,-180,-170,-160,-147,-140,-130,-120,-110,-80,-50,-49,-45,-39,-33,-26,-21,-18,-17,-19,-22,-22,-26,-27,-25,-22,-16,-9,-3,2,6,6,4,1,1,-3,-4,-2,2,7,14,20,26,29,30,28,24,24,21,20,21,25,31,37,44,49,50,50,80];
      | B=[-41.5,-41.5,-63,-20,-63,-20,-63,-20,-41.5,-41.5,-41.5,-34,-26,-21,-20,-22,-28,-37,-47,-57,-63,-63,-54,-44,-34,-26,-21,-20,-22,-28,-37,-47,-57,-63,-63,-54,-44,-34,-26,-21,-20,-22,-28,-37,-47,-57,-63,-63,-54,-44,-34,-26,-21,-20,-22,-28,-37,-41.50,-41.5];
      | plot(A,B);
      | color('black');
      | port_label('LConn', 1, '+')
  38 : Subsystem
  38 Y I : Subsystem  mask(Single Phase ZIP Load){Vnom=1.0*2401.78, fnom=60, Pnom=20e3*a, Qnom=10e3*a, LoadType=constant I, Vlim=0.7}
      mask prompts: Vnom "Nominal Voltage Vn (Vrms)"; fnom "Nominal Frequency fn (Hz)"; Pnom "Nominal Active power (W)"; Qnom "Nominal Reactive power (VAR)"; LoadType "Load Type"; Vlim "Minimum voltage (pu)"
      mask help:
      | Notes:
      | Single Phase ZIP load model which gets converted to constant Z type if the voltage becomes lower than the Minimum Voltage.
      mask TypeOptions LoadType: Constant Z | constant I | constant P
      mask DialogControl ParameterTabVar0 Prompt: Parameters
      mask DialogControl ParameterTabVar1 Prompt: Type
      mask Display:
      | color('red');
      | A=[-210,-180,-170,-160,-147,-140,-130,-120,-110,-80,-50,-49,-45,-39,-33,-26,-21,-18,-17,-19,-22,-22,-26,-27,-25,-22,-16,-9,-3,2,6,6,4,1,1,-3,-4,-2,2,7,14,20,26,29,30,28,24,24,21,20,21,25,31,37,44,49,50,50,80];
      | B=[-41.5,-41.5,-63,-20,-63,-20,-63,-20,-41.5,-41.5,-41.5,-34,-26,-21,-20,-22,-28,-37,-47,-57,-63,-63,-54,-44,-34,-26,-21,-20,-22,-28,-37,-47,-57,-63,-63,-54,-44,-34,-26,-21,-20,-22,-28,-37,-47,-57,-63,-63,-54,-44,-34,-26,-21,-20,-22,-28,-37,-41.50,-41.5];
      | plot(A,B);
      | color('black');
      | port_label('LConn', 1, '+')
  38-39 10 : powerlib/Elements/Distributed Parameters Line  Phases=1  Frequency=60  Resistance=R_10(2,2)  Inductance=L_10(2,2)  Capacitance=C_10(2,2)  Length=325*ft2km  x1=[3416.97117543852;376.991118430775;-2.09716413717725]  x2=[3416.97093529354;376.991118430775;-2.0971642314999]  x3=[6.25354813426528;376.991118430775;-2.0973161232589]  x4=[6.26038105220899;376.991118430775;-2.09716423149761]  x5=4.02920507104677e-07  V1=[2.049e+04;377;-2.115]  V2=[2.048e+04;377;-2.115]  I1=[33.62;377;-2.106]  I2=[35.2;377;-2.126]  nHarmo=1  Measurements=None
      settings: SourceProductName=Simscape Electrical
  39 : Subsystem
  39 Y PQ : Subsystem  mask(Single Phase ZIP Load){Vnom=1.0*2401.78, fnom=60, Pnom=20e3*a, Qnom=10e3*a, LoadType=constant P, Vlim=0.7}
      mask prompts: Vnom "Nominal Voltage Vn (Vrms)"; fnom "Nominal Frequency fn (Hz)"; Pnom "Nominal Active power (W)"; Qnom "Nominal Reactive power (VAR)"; LoadType "Load Type"; Vlim "Minimum voltage (pu)"
      mask help:
      | Notes:
      | Single Phase ZIP load model which gets converted to constant Z type if the voltage becomes lower than the Minimum Voltage.
      mask TypeOptions LoadType: Constant Z | constant I | constant P
      mask DialogControl ParameterTabVar0 Prompt: Parameters
      mask DialogControl ParameterTabVar1 Prompt: Type
      mask Display:
      | color('red');
      | A=[-210,-180,-170,-160,-147,-140,-130,-120,-110,-80,-50,-49,-45,-39,-33,-26,-21,-18,-17,-19,-22,-22,-26,-27,-25,-22,-16,-9,-3,2,6,6,4,1,1,-3,-4,-2,2,7,14,20,26,29,30,28,24,24,21,20,21,25,31,37,44,49,50,50,80];
      | B=[-41.5,-41.5,-63,-20,-63,-20,-63,-20,-41.5,-41.5,-41.5,-34,-26,-21,-20,-22,-28,-37,-47,-57,-63,-63,-54,-44,-34,-26,-21,-20,-22,-28,-37,-47,-57,-63,-63,-54,-44,-34,-26,-21,-20,-22,-28,-37,-47,-57,-63,-63,-54,-44,-34,-26,-21,-20,-22,-28,-37,-41.50,-41.5];
      | plot(A,B);
      | color('black');
      | port_label('LConn', 1, '+')
  4 : Subsystem
  40 : powerlib/Measurements/Three-Phase V-I Measurement  VoltageMeasurement=phase-to-ground  SetLabelV=on  LabelV=V40  Vpu=off  VpuLL=off  CurrentMeasurement=no  SetLabelI=on  LabelI=I800  Ipu=off  Pbase=100e6  Vbase=24900  OutputType=Complex  PhasorSimulation=on  PSBequivalent=0
      settings: SourceProductName=Simscape Electrical
  40-41 11 : powerlib/Elements/Distributed Parameters Line  Phases=1  Frequency=60  Resistance=R_11(3,3)  Inductance=L_11(3,3)  Capacitance=C_11(3,3)  Length=325*ft2km  x1=[3419.45252901836;376.991118430775;2.09156955130138]  x2=[3419.45228869973;376.991118430775;2.09156945697807]  x3=[6.25808935868782;376.991118430775;2.091417562353]  x4=[6.26492725680185;376.991118430775;2.09156945984391]  x5=4.02920507104677e-07  V1=[2.049e+04;377;-2.115]  V2=[2.048e+04;377;-2.115]  I1=[33.62;377;-2.106]  I2=[35.2;377;-2.126]  nHarmo=1  Measurements=None
      settings: SourceProductName=Simscape Electrical
  40-42 1 : powerlib/Elements/Distributed Parameters Line  Phases=3  Frequency=60  Resistance=R_1  Inductance=L_1  Capacitance=C_1  Length=250*ft2km  x1=[437.491775418153 4182.75150382427 4186.35948826417;376.991118430775 376.991118430775 376.991118430775;1.69003309652954 -2.40522189116136 2.30714358685808]  x2=[437.491191443315 4182.75145447974 4186.35968944777;376.991118430775 376.991118430775 376.991118430775;1.69003359891336 -2.40522205110213 2.30714336369219]  x3=[0.574920993489203 15.5928430286635 12.3179645674927;376.991118430775 376.991118430775 376.991118430775;1.70117238149111 -2.40586952349109 2.30584071870096]  x4=[0.575198543256048 15.633467378587 12.3608717558467;376.991118430775 376.991118430775 376.991118430775;1.67878151536702 -2.40467404486045 2.30834423521702]  x5=3.13537493203638e-07  V1=ones(3,3)  V2=ones(3,3)  I1=ones(3,3)  I2=ones(3,3)  nHarmo=1  Measurements=None
      settings: SourceProductName=Simscape Electrical
  41 : Subsystem
  41 Y PQ : Subsystem  mask(Single Phase ZIP Load){Vnom=1.0*2401.78, fnom=60, Pnom=20e3*a, Qnom=10e3*a, LoadType=constant P, Vlim=0.7}
      mask prompts: Vnom "Nominal Voltage Vn (Vrms)"; fnom "Nominal Frequency fn (Hz)"; Pnom "Nominal Active power (W)"; Qnom "Nominal Reactive power (VAR)"; LoadType "Load Type"; Vlim "Minimum voltage (pu)"
      mask help:
      | Notes:
      | Single Phase ZIP load model which gets converted to constant Z type if the voltage becomes lower than the Minimum Voltage.
      mask TypeOptions LoadType: Constant Z | constant I | constant P
      mask DialogControl ParameterTabVar0 Prompt: Parameters
      mask DialogControl ParameterTabVar1 Prompt: Type
      mask Display:
      | color('red');
      | A=[-210,-180,-170,-160,-147,-140,-130,-120,-110,-80,-50,-49,-45,-39,-33,-26,-21,-18,-17,-19,-22,-22,-26,-27,-25,-22,-16,-9,-3,2,6,6,4,1,1,-3,-4,-2,2,7,14,20,26,29,30,28,24,24,21,20,21,25,31,37,44,49,50,50,80];
      | B=[-41.5,-41.5,-63,-20,-63,-20,-63,-20,-41.5,-41.5,-41.5,-34,-26,-21,-20,-22,-28,-37,-47,-57,-63,-63,-54,-44,-34,-26,-21,-20,-22,-28,-37,-47,-57,-63,-63,-54,-44,-34,-26,-21,-20,-22,-28,-37,-47,-57,-63,-63,-54,-44,-34,-26,-21,-20,-22,-28,-37,-41.50,-41.5];
      | plot(A,B);
      | color('black');
      | port_label('LConn', 1, '+')
  4160 V swing : powerlib/Electrical Sources/Three-Phase Source  InternalConnection=Yg  VoltagePhases=on  Voltage=120e3  PhaseAngle=0  Voltage_phases=[1.0 1.0 1.0]*4160/sqrt(3)  PhaseAngles_phases=[0 -120 120 ]  Frequency=60  NonIdealSource=off  SpecifyImpedance=on  Resistance=.0001  Inductance=16.58e-3  ShortCircuitLevel=10e6  BaseVoltage=4160  XRratio=4.67e4  BusType=swing  Pref=0  Qref=0  Prefabc=[4e6/3 4e6/3 4e6/3]  Qrefabc=[0 0 0]  Qmin="[-inf  -inf -inf]"  Qmax="[inf  inf inf]"
      settings: SourceProductName=Simscape Electrical
  42 : powerlib/Measurements/Three-Phase V-I Measurement  VoltageMeasurement=phase-to-ground  SetLabelV=on  LabelV=V42  Vpu=off  VpuLL=off  CurrentMeasurement=no  SetLabelI=on  LabelI=I800  Ipu=off  Pbase=100e6  Vbase=24900  OutputType=Complex  PhasorSimulation=on  PSBequivalent=0
      settings: SourceProductName=Simscape Electrical
  42 Y PQ : Subsystem  mask(Single Phase ZIP Load){Vnom=1.0*2401.78, fnom=60, Pnom=20e3*a, Qnom=10e3*a, LoadType=constant P, Vlim=0.7}
      mask prompts: Vnom "Nominal Voltage Vn (Vrms)"; fnom "Nominal Frequency fn (Hz)"; Pnom "Nominal Active power (W)"; Qnom "Nominal Reactive power (VAR)"; LoadType "Load Type"; Vlim "Minimum voltage (pu)"
      mask help:
      | Notes:
      | Single Phase ZIP load model which gets converted to constant Z type if the voltage becomes lower than the Minimum Voltage.
      mask TypeOptions LoadType: Constant Z | constant I | constant P
      mask DialogControl ParameterTabVar0 Prompt: Parameters
      mask DialogControl ParameterTabVar1 Prompt: Type
      mask Display:
      | color('red');
      | A=[-210,-180,-170,-160,-147,-140,-130,-120,-110,-80,-50,-49,-45,-39,-33,-26,-21,-18,-17,-19,-22,-22,-26,-27,-25,-22,-16,-9,-3,2,6,6,4,1,1,-3,-4,-2,2,7,14,20,26,29,30,28,24,24,21,20,21,25,31,37,44,49,50,50,80];
      | B=[-41.5,-41.5,-63,-20,-63,-20,-63,-20,-41.5,-41.5,-41.5,-34,-26,-21,-20,-22,-28,-37,-47,-57,-63,-63,-54,-44,-34,-26,-21,-20,-22,-28,-37,-47,-57,-63,-63,-54,-44,-34,-26,-21,-20,-22,-28,-37,-47,-57,-63,-63,-54,-44,-34,-26,-21,-20,-22,-28,-37,-41.50,-41.5];
      | plot(A,B);
      | color('black');
      | port_label('LConn', 1, '+')
  42-43 10 : powerlib/Elements/Distributed Parameters Line  Phases=1  Frequency=60  Resistance=R_10(2,2)  Inductance=L_10(2,2)  Capacitance=C_10(2,2)  Length=500*ft2km  x1=[3416.97220032656;376.991118430775;-2.09724574237351]  x2=[3416.97186352866;376.991118430775;-2.09724589691147]  x3=[6.25317166811513;376.991118430775;-2.09747957052881]  x4=[6.26000400881998;376.991118430775;-2.09724589819975]  x5=6.19877703237964e-07  V1=[2.049e+04;377;-2.115]  V2=[2.048e+04;377;-2.115]  I1=[33.62;377;-2.106]  I2=[35.2;377;-2.126]  nHarmo=1  Measurements=None
      settings: SourceProductName=Simscape Electrical
  42-44 1 : powerlib/Elements/Distributed Parameters Line  Phases=3  Frequency=60  Resistance=R_1  Inductance=L_1  Capacitance=C_1  Length=200*ft2km  x1=[437.491191443315 4182.75145447974 4186.35968944777;376.991118430775 376.991118430775 376.991118430775;1.69005723908341 -2.40520243720617 2.30716289227553]  x2=[437.490759011172 4182.75141517735 4186.35982793965;376.991118430775 376.991118430775 376.991118430775;1.69005716862642 -2.40520254080512 2.30716273195441]  x3=[0.572603128623654 15.5966866943866 12.3201466095295;376.991118430775 376.991118430775 376.991118430775;1.69879332184654 -2.4057090388268 2.30601344693565]  x4=[0.577495163592198 15.6298747186743 12.3588444514311;376.991118430775 376.991118430775 376.991118430775;1.68130093146124 -2.40477538791447 2.30823058571298]  x5=2.50829994562911e-07  V1=ones(3,3)  V2=ones(3,3)  I1=ones(3,3)  I2=ones(3,3)  nHarmo=1  Measurements=None
      settings: SourceProductName=Simscape Electrical
  43 : Subsystem
  43 Y Z : Subsystem  mask(Single Phase ZIP Load){Vnom=1.0*2401.78, fnom=60, Pnom=40e3*a, Qnom=20e3*a, LoadType=Constant Z, Vlim=0.7}
      mask prompts: Vnom "Nominal Voltage Vn (Vrms)"; fnom "Nominal Frequency fn (Hz)"; Pnom "Nominal Active power (W)"; Qnom "Nominal Reactive power (VAR)"; LoadType "Load Type"; Vlim "Minimum voltage (pu)"
      mask help:
      | Notes:
      | Single Phase ZIP load model which gets converted to constant Z type if the voltage becomes lower than the Minimum Voltage.
      mask TypeOptions LoadType: Constant Z | constant I | constant P
      mask DialogControl ParameterTabVar0 Prompt: Parameters
      mask DialogControl ParameterTabVar1 Prompt: Type
      mask Display:
      | color('red');
      | A=[-210,-180,-170,-160,-147,-140,-130,-120,-110,-80,-50,-49,-45,-39,-33,-26,-21,-18,-17,-19,-22,-22,-26,-27,-25,-22,-16,-9,-3,2,6,6,4,1,1,-3,-4,-2,2,7,14,20,26,29,30,28,24,24,21,20,21,25,31,37,44,49,50,50,80];
      | B=[-41.5,-41.5,-63,-20,-63,-20,-63,-20,-41.5,-41.5,-41.5,-34,-26,-21,-20,-22,-28,-37,-47,-57,-63,-63,-54,-44,-34,-26,-21,-20,-22,-28,-37,-47,-57,-63,-63,-54,-44,-34,-26,-21,-20,-22,-28,-37,-47,-57,-63,-63,-54,-44,-34,-26,-21,-20,-22,-28,-37,-41.50,-41.5];
      | plot(A,B);
      | color('black');
      | port_label('LConn', 1, '+')
  44 : powerlib/Measurements/Three-Phase V-I Measurement  VoltageMeasurement=phase-to-ground  SetLabelV=on  LabelV=V44  Vpu=off  VpuLL=off  CurrentMeasurement=no  SetLabelI=on  LabelI=I800  Ipu=off  Pbase=100e6  Vbase=24900  OutputType=Complex  PhasorSimulation=on  PSBequivalent=0
      settings: SourceProductName=Simscape Electrical
  44-45 9 : powerlib/Elements/Distributed Parameters Line  Phases=1  Frequency=60  Resistance=R_9(1,1)  Inductance=L_9(1,1)  Capacitance=C_9(1,1)  Length=200*ft2km  x1=[3417.75961772403;376.991118430775;-0.00431515833539889]  x2=[3417.75933329084;376.991118430775;-0.00431527765636545]  x3=[6.25184400963475;376.991118430775;-0.00454910343251728]  x4=[6.26551375996762;376.991118430775;-0.00417521837510541]  x5=2.47951081295186e-07  V1=[2.049e+04;377;-2.115]  V2=[2.048e+04;377;-2.115]  I1=[33.62;377;-2.106]  I2=[35.2;377;-2.126]  nHarmo=1  Measurements=None
      settings: SourceProductName=Simscape Electrical
  44-47 1 : powerlib/Elements/Distributed Parameters Line  Phases=3  Frequency=60  Resistance=R_1  Inductance=L_1  Capacitance=C_1  Length=250*ft2km  x1=[437.490759011172 4182.75141517735 4186.35982793965;376.991118430775 376.991118430775 376.991118430775;1.69003352845638 -2.40522215470108 2.30714320337107]  x2=[437.490590885662 4182.75143220358 4186.35987584691;376.991118430775 376.991118430775 376.991118430775;1.69003318362945 -2.40522226486562 2.30714303603046]  x3=[0.57293263079376 15.5999849565492 12.3221854687659;376.991118430775 376.991118430775 376.991118430775;1.69177314687777 -2.40577870981539 2.30636613905012]  x4=[0.577114552046216 15.6263234721165 12.3566395949364;376.991118430775 376.991118430775 376.991118430775;1.68818839818531 -2.40476463590446 2.30782042606138]  x5=3.13537493203638e-07  V1=ones(3,3)  V2=ones(3,3)  I1=ones(3,3)  I2=ones(3,3)  nHarmo=1  Measurements=None
      settings: SourceProductName=Simscape Electrical
  45 : Subsystem
  45 Y I : Subsystem  mask(Single Phase ZIP Load){Vnom=1.0*2401.78, fnom=60, Pnom=20e3*a, Qnom=10e3*a, LoadType=constant I, Vlim=0.7}
      mask prompts: Vnom "Nominal Voltage Vn (Vrms)"; fnom "Nominal Frequency fn (Hz)"; Pnom "Nominal Active power (W)"; Qnom "Nominal Reactive power (VAR)"; LoadType "Load Type"; Vlim "Minimum voltage (pu)"
      mask help:
      | Notes:
      | Single Phase ZIP load model which gets converted to constant Z type if the voltage becomes lower than the Minimum Voltage.
      mask TypeOptions LoadType: Constant Z | constant I | constant P
      mask DialogControl ParameterTabVar0 Prompt: Parameters
      mask DialogControl ParameterTabVar1 Prompt: Type
      mask Display:
      | color('red');
      | A=[-210,-180,-170,-160,-147,-140,-130,-120,-110,-80,-50,-49,-45,-39,-33,-26,-21,-18,-17,-19,-22,-22,-26,-27,-25,-22,-16,-9,-3,2,6,6,4,1,1,-3,-4,-2,2,7,14,20,26,29,30,28,24,24,21,20,21,25,31,37,44,49,50,50,80];
      | B=[-41.5,-41.5,-63,-20,-63,-20,-63,-20,-41.5,-41.5,-41.5,-34,-26,-21,-20,-22,-28,-37,-47,-57,-63,-63,-54,-44,-34,-26,-21,-20,-22,-28,-37,-47,-57,-63,-63,-54,-44,-34,-26,-21,-20,-22,-28,-37,-47,-57,-63,-63,-54,-44,-34,-26,-21,-20,-22,-28,-37,-41.50,-41.5];
      | plot(A,B);
      | color('black');
      | port_label('LConn', 1, '+')
  45-46 9 : powerlib/Elements/Distributed Parameters Line  Phases=1  Frequency=60  Resistance=R_9(1,1)  Inductance=L_9(1,1)  Capacitance=C_9(1,1)  Length=300*ft2km  x1=[3417.75933329084;376.991118430775;-0.00436201533409225]  x2=[3417.75910876776;376.991118430775;-0.00436210159312945]  x3=[6.25504464510249;376.991118430775;-0.00450230978297983]  x4=[6.26187921797813;376.991118430775;-0.00436210158141976]  x5=3.71926621942778e-07  V1=[2.049e+04;377;-2.115]  V2=[2.048e+04;377;-2.115]  I1=[33.62;377;-2.106]  I2=[35.2;377;-2.126]  nHarmo=1  Measurements=None
      settings: SourceProductName=Simscape Electrical
  450 : powerlib/Measurements/Three-Phase V-I Measurement  VoltageMeasurement=phase-to-ground  SetLabelV=on  LabelV=V450  Vpu=off  VpuLL=off  CurrentMeasurement=no  SetLabelI=on  LabelI=I65  Ipu=off  Pbase=100e6  Vbase=24900  OutputType=Complex  PhasorSimulation=on  PSBequivalent=0
      settings: SourceProductName=Simscape Electrical
  450-451 : powerlib/Elements/Three-Phase Breaker  InitialState=open  SwitchA=off  SwitchB=off  SwitchC=off  SwitchTimes="[1/60  5/60]"  External=off  BreakerResistance=0.01  SnubberResistance=1e6  SnubberCapacitance=inf  Measurements=None
      settings: SourceProductName=Simscape Electrical
  46 : Subsystem
  46 Y PQ : Subsystem  mask(Single Phase ZIP Load){Vnom=1.0*2401.78, fnom=60, Pnom=20e3*a, Qnom=10e3*a, LoadType=constant P, Vlim=0.7}
      mask prompts: Vnom "Nominal Voltage Vn (Vrms)"; fnom "Nominal Frequency fn (Hz)"; Pnom "Nominal Active power (W)"; Qnom "Nominal Reactive power (VAR)"; LoadType "Load Type"; Vlim "Minimum voltage (pu)"
      mask help:
      | Notes:
      | Single Phase ZIP load model which gets converted to constant Z type if the voltage becomes lower than the Minimum Voltage.
      mask TypeOptions LoadType: Constant Z | constant I | constant P
      mask DialogControl ParameterTabVar0 Prompt: Parameters
      mask DialogControl ParameterTabVar1 Prompt: Type
      mask Display:
      | color('red');
      | A=[-210,-180,-170,-160,-147,-140,-130,-120,-110,-80,-50,-49,-45,-39,-33,-26,-21,-18,-17,-19,-22,-22,-26,-27,-25,-22,-16,-9,-3,2,6,6,4,1,1,-3,-4,-2,2,7,14,20,26,29,30,28,24,24,21,20,21,25,31,37,44,49,50,50,80];
      | B=[-41.5,-41.5,-63,-20,-63,-20,-63,-20,-41.5,-41.5,-41.5,-34,-26,-21,-20,-22,-28,-37,-47,-57,-63,-63,-54,-44,-34,-26,-21,-20,-22,-28,-37,-47,-57,-63,-63,-54,-44,-34,-26,-21,-20,-22,-28,-37,-47,-57,-63,-63,-54,-44,-34,-26,-21,-20,-22,-28,-37,-41.50,-41.5];
      | plot(A,B);
      | color('black');
      | port_label('LConn', 1, '+')
  47 : powerlib/Measurements/Three-Phase V-I Measurement  VoltageMeasurement=phase-to-ground  SetLabelV=on  LabelV=V47  Vpu=off  VpuLL=off  CurrentMeasurement=no  SetLabelI=on  LabelI=I800  Ipu=off  Pbase=100e6  Vbase=24900  OutputType=Complex  PhasorSimulation=on  PSBequivalent=0
      settings: SourceProductName=Simscape Electrical
  47 Y I : Subsystem  mask(Three Phase Star ZIP Load (Phasor)){Vnom=4160, fnom=60, Pnom=[35 35 35 ]*1e3*a, Qnom=[25 25 25 ]*1e3*a, LoadType=Constant I, Vlim=0.7}
      mask prompts: Vnom "Nominal Ph-Ph voltage (Vrms)"; fnom "Nominal Frequency fn (Hz)"; Pnom "Nominal Per Phase Active Power [Pa Pb Pc] (W)"; Qnom "Nominal Per Phase Reactive Power [Qa Qb Qc] (VAR)"; LoadType "Load Type"; Vlim "Minimum voltage (pu)"
      mask help:
      | Notes:
      | Three Phase Star Connected ZIP load model which gets converted to constant Z type if the voltage becomes lower than the Minimum Voltage.
      mask TypeOptions LoadType: Constant Z | Constant I | Constant P
      mask DialogControl ParameterTabVar0 Prompt: Parameters
      mask DialogControl ParameterTabVar01 Prompt: Type
      mask Display:
      | color('red');
      | %load figure 0deg
      | A=[-210,-180,-170,-160,-147,-140,-130,-120,-110,-80,-50,-49,-45,-39,-33,-26,-21,-18,-17,-19,-22,-22,-26,-27,-25,-22,-16,-9,-3,2,6,6,4,1,1,-3,-4,-2,2,7,14,20,26,29,30,28,24,24,21,20,21,25,31,37,44,49,50,50,80];
      | B=[-41.5,-41.5,-63,-20,-63,-20,-63,-20,-41.5,-41.5,-41.5,-34,-26,-21,-20,-22,-28,-37,-47,-57,-63,-63,-54,-44,-34,-26,-21,-20,-22,-28,-37,-47,-57,-63,-63,-54,-44,-34,-26,-21,-20,-22,-28,-37,-47,-57,-63,-63,-54,-44,-34,-26,-21,-20,-22,-28,-37,-41.50,-41.5];
      | % plot(A,B);
      | 
      | %load figure 0deg inverted
      | A1=[-80,-50,-49,-45,-39,-33,-26,-21,-18,-17,-19,-22,-22,-26,-27,-25,-22,-16,-9,-3,2,6,6,4,1,1,-3,-4,-2,2,7,14,20,26,29,30,28,24,24,21,20,21,25,31,37,44,49,50,50,80,110,120,130,143,150,160,170,180,210];
      | B1=[-41.5,-41.5,-34,-26,-21,-20,-22,-28,-37,-47,-57,-63,-63,-54,-44,-34,-26,-21,-20,-22,-28,-37,-47,-57,-63,-63,-54,-44,-34,-26,-21,-20,-22,-28,-37,-47,-57,-63,-63,-54,-44,-34,-26,-21,-20,-22,-28,-37,-41.5,-41.5,-41.5,-63,-20,-63,-20,-63,-20,-41.5,-41.5];
      | 
      | 
      | %load figure 90deg
      | C=[-41.5,-41.5,-20,-63,-20,-63,-20,-63,-41.5,-41.5,-41.5,-37,-28,-22,-20,-21,-26,-34,-44,-54,-63,-63,-57,-47,-37,-28,-22,-20,-21,-26,-34,-44,-54,-63,-63,-57,-47,-37,-28,-22,-20,-21,-26,-34,-44,-54,-63,-63,-57,-47,-37,-28,-22,-20,-21,-26,-34,-41.5,-41.5];
      | D=[190,160,150,140,130,123,110,100,90,80,50,50,49,44,37,31,25,21,20,21,24,24,28,30,29,26,20,14,7,2,-2,-4,-3,1,1,4,6,6,2,-3,-9,-16,-22,-25,-27,-26,-22,-22,-19,-17,-18,-21,-26,-33,-39,-45,-49,-50,-70];
      | plot(C,D);
      | 
      | 
      | %load figure -120deg
      | c=1*exp(sqrt(-1)*(-60*pi/180));
      | l=A1+j*B1;
      | m=l*c;
      | E=real(m);F=imag(m);
      | E=E+34.4400;F=F-118.53;
      | plot(E,F);
      | 
      | %load figure +120deg
      | c=1*exp(sqrt(-1)*(60*pi/180));
      | l=A+j*B;
      | m=l*c;
      | G=real(m);
      | H=imag(m);
      | G=G-117.44;H=H-118.5300;
      | plot(G,H);
      | 
      | color('black');
      | port_label('LConn', 1, 'A')
      | port_label('LConn', 2, 'B')
      | port_label('LConn', 3, 'C')
  47-48 4 : powerlib/Elements/Distributed Parameters Line  Phases=3  Frequency=60  Resistance=R_4  Inductance=L_4  Capacitance=C_4  Length=150*ft2km  x1=[438.082259281131 4184.31860585284 4184.78613460211;376.991118430775 376.991118430775 376.991118430775;0.395204232321518 -0.219930683913646 -1.78937685432451]  x2=[438.082306710962 4184.3186077851 4184.7861906173;376.991118430775 376.991118430775 376.991118430775;0.395203941368649 -0.219930753150724 -1.78937691015084]  x3=[0.574079595263843 12.3213477629886 15.6111469587997;376.991118430775 376.991118430775 376.991118430775;0.392427775637933 -0.220400628597507 -1.78998240194141]  x4=[0.577541599805126 12.345755578495 15.6308602416168;376.991118430775 376.991118430775 376.991118430775;0.397893047274991 -0.219520265693626 -1.78883093126267]  x5=1.88122495922183e-07  V1=ones(3,3)  V2=ones(3,3)  I1=ones(3,3)  I2=ones(3,3)  nHarmo=1  Measurements=None
      settings: SourceProductName=Simscape Electrical
  47-49 4 : powerlib/Elements/Distributed Parameters Line  Phases=3  Frequency=60  Resistance=R_4  Inductance=L_4  Capacitance=C_4  Length=250*ft2km  x1=[438.082306710962 4184.3186077851 4184.7861906173;376.991118430775 376.991118430775 376.991118430775;0.395156661028556 -0.219969810317401 -1.78941613794274]  x2=[438.082381973315 4184.31863980955 4184.78631236162;376.991118430775 376.991118430775 376.991118430775;0.395156193508634 -0.219969889248016 -1.78941620047031]  x3=[0.574129805201193 12.3253763938985 15.6150760021422;376.991118430775 376.991118430775 376.991118430775;0.392470972321537 -0.220381282237884 -1.78996249328575]  x4=[0.577474818811235 12.3414106146189 15.6264232668842;376.991118430775 376.991118430775 376.991118430775;0.397708466821702 -0.219656532397612 -1.78896827704495]  x5=3.13537493203638e-07  V1=ones(3,3)  V2=ones(3,3)  I1=ones(3,3)  I2=ones(3,3)  nHarmo=1  Measurements=None
      settings: SourceProductName=Simscape Electrical
  48 : powerlib/Measurements/Three-Phase V-I Measurement  VoltageMeasurement=phase-to-ground  SetLabelV=on  LabelV=V48  Vpu=off  VpuLL=off  CurrentMeasurement=no  SetLabelI=on  LabelI=I800  Ipu=off  Pbase=100e6  Vbase=24900  OutputType=Complex  PhasorSimulation=on  PSBequivalent=0
      settings: SourceProductName=Simscape Electrical
  48 Y Z : Subsystem  mask(Three Phase Star ZIP Load (Phasor)){Vnom=4160, fnom=60, Pnom=[70 70 70]*1e3*a, Qnom=[50 50 50]*1e3*a, LoadType=Constant Z, Vlim=0.7}
      mask prompts: Vnom "Nominal Ph-Ph voltage (Vrms)"; fnom "Nominal Frequency fn (Hz)"; Pnom "Nominal Per Phase Active Power [Pa Pb Pc] (W)"; Qnom "Nominal Per Phase Reactive Power [Qa Qb Qc] (VAR)"; LoadType "Load Type"; Vlim "Minimum voltage (pu)"
      mask help:
      | Notes:
      | Three Phase Star Connected ZIP load model which gets converted to constant Z type if the voltage becomes lower than the Minimum Voltage.
      mask TypeOptions LoadType: Constant Z | Constant I | Constant P
      mask DialogControl ParameterTabVar0 Prompt: Parameters
      mask DialogControl ParameterTabVar01 Prompt: Type
      mask Display:
      | color('red');
      | %load figure 0deg
      | A=[-210,-180,-170,-160,-147,-140,-130,-120,-110,-80,-50,-49,-45,-39,-33,-26,-21,-18,-17,-19,-22,-22,-26,-27,-25,-22,-16,-9,-3,2,6,6,4,1,1,-3,-4,-2,2,7,14,20,26,29,30,28,24,24,21,20,21,25,31,37,44,49,50,50,80];
      | B=[-41.5,-41.5,-63,-20,-63,-20,-63,-20,-41.5,-41.5,-41.5,-34,-26,-21,-20,-22,-28,-37,-47,-57,-63,-63,-54,-44,-34,-26,-21,-20,-22,-28,-37,-47,-57,-63,-63,-54,-44,-34,-26,-21,-20,-22,-28,-37,-47,-57,-63,-63,-54,-44,-34,-26,-21,-20,-22,-28,-37,-41.50,-41.5];
      | % plot(A,B);
      | 
      | %load figure 0deg inverted
      | A1=[-80,-50,-49,-45,-39,-33,-26,-21,-18,-17,-19,-22,-22,-26,-27,-25,-22,-16,-9,-3,2,6,6,4,1,1,-3,-4,-2,2,7,14,20,26,29,30,28,24,24,21,20,21,25,31,37,44,49,50,50,80,110,120,130,143,150,160,170,180,210];
      | B1=[-41.5,-41.5,-34,-26,-21,-20,-22,-28,-37,-47,-57,-63,-63,-54,-44,-34,-26,-21,-20,-22,-28,-37,-47,-57,-63,-63,-54,-44,-34,-26,-21,-20,-22,-28,-37,-47,-57,-63,-63,-54,-44,-34,-26,-21,-20,-22,-28,-37,-41.5,-41.5,-41.5,-63,-20,-63,-20,-63,-20,-41.5,-41.5];
      | 
      | 
      | %load figure 90deg
      | C=[-41.5,-41.5,-20,-63,-20,-63,-20,-63,-41.5,-41.5,-41.5,-37,-28,-22,-20,-21,-26,-34,-44,-54,-63,-63,-57,-47,-37,-28,-22,-20,-21,-26,-34,-44,-54,-63,-63,-57,-47,-37,-28,-22,-20,-21,-26,-34,-44,-54,-63,-63,-57,-47,-37,-28,-22,-20,-21,-26,-34,-41.5,-41.5];
      | D=[190,160,150,140,130,123,110,100,90,80,50,50,49,44,37,31,25,21,20,21,24,24,28,30,29,26,20,14,7,2,-2,-4,-3,1,1,4,6,6,2,-3,-9,-16,-22,-25,-27,-26,-22,-22,-19,-17,-18,-21,-26,-33,-39,-45,-49,-50,-70];
      | plot(C,D);
      | 
      | 
      | %load figure -120deg
      | c=1*exp(sqrt(-1)*(-60*pi/180));
      | l=A1+j*B1;
      | m=l*c;
      | E=real(m);F=imag(m);
      | E=E+34.4400;F=F-118.53;
      | plot(E,F);
      | 
      | %load figure +120deg
      | c=1*exp(sqrt(-1)*(60*pi/180));
      | l=A+j*B;
      | m=l*c;
      | G=real(m);
      | H=imag(m);
      | G=G-117.44;H=H-118.5300;
      | plot(G,H);
      | 
      | color('black');
      | port_label('LConn', 1, 'A')
      | port_label('LConn', 2, 'B')
      | port_label('LConn', 3, 'C')
  49 : powerlib/Measurements/Three-Phase V-I Measurement  VoltageMeasurement=phase-to-ground  SetLabelV=on  LabelV=V49  Vpu=off  VpuLL=off  CurrentMeasurement=no  SetLabelI=on  LabelI=I800  Ipu=off  Pbase=100e6  Vbase=24900  OutputType=Complex  PhasorSimulation=on  PSBequivalent=0
      settings: SourceProductName=Simscape Electrical
  49 Y PQ : Subsystem  mask(Three Phase Star ZIP Load (Phasor)){Vnom=4160, fnom=60, Pnom=[35 70 35]*1e3*a, Qnom=[25 50 20]*1e3*a, LoadType=Constant P, Vlim=0.7}
      mask prompts: Vnom "Nominal Ph-Ph voltage (Vrms)"; fnom "Nominal Frequency fn (Hz)"; Pnom "Nominal Per Phase Active Power [Pa Pb Pc] (W)"; Qnom "Nominal Per Phase Reactive Power [Qa Qb Qc] (VAR)"; LoadType "Load Type"; Vlim "Minimum voltage (pu)"
      mask help:
      | Notes:
      | Three Phase Star Connected ZIP load model which gets converted to constant Z type if the voltage becomes lower than the Minimum Voltage.
      mask TypeOptions LoadType: Constant Z | Constant I | Constant P
      mask DialogControl ParameterTabVar0 Prompt: Parameters
      mask DialogControl ParameterTabVar01 Prompt: Type
      mask Display:
      | color('red');
      | %load figure 0deg
      | A=[-210,-180,-170,-160,-147,-140,-130,-120,-110,-80,-50,-49,-45,-39,-33,-26,-21,-18,-17,-19,-22,-22,-26,-27,-25,-22,-16,-9,-3,2,6,6,4,1,1,-3,-4,-2,2,7,14,20,26,29,30,28,24,24,21,20,21,25,31,37,44,49,50,50,80];
      | B=[-41.5,-41.5,-63,-20,-63,-20,-63,-20,-41.5,-41.5,-41.5,-34,-26,-21,-20,-22,-28,-37,-47,-57,-63,-63,-54,-44,-34,-26,-21,-20,-22,-28,-37,-47,-57,-63,-63,-54,-44,-34,-26,-21,-20,-22,-28,-37,-47,-57,-63,-63,-54,-44,-34,-26,-21,-20,-22,-28,-37,-41.50,-41.5];
      | % plot(A,B);
      | 
      | %load figure 0deg inverted
      | A1=[-80,-50,-49,-45,-39,-33,-26,-21,-18,-17,-19,-22,-22,-26,-27,-25,-22,-16,-9,-3,2,6,6,4,1,1,-3,-4,-2,2,7,14,20,26,29,30,28,24,24,21,20,21,25,31,37,44,49,50,50,80,110,120,130,143,150,160,170,180,210];
      | B1=[-41.5,-41.5,-34,-26,-21,-20,-22,-28,-37,-47,-57,-63,-63,-54,-44,-34,-26,-21,-20,-22,-28,-37,-47,-57,-63,-63,-54,-44,-34,-26,-21,-20,-22,-28,-37,-47,-57,-63,-63,-54,-44,-34,-26,-21,-20,-22,-28,-37,-41.5,-41.5,-41.5,-63,-20,-63,-20,-63,-20,-41.5,-41.5];
      | 
      | 
      | %load figure 90deg
      | C=[-41.5,-41.5,-20,-63,-20,-63,-20,-63,-41.5,-41.5,-41.5,-37,-28,-22,-20,-21,-26,-34,-44,-54,-63,-63,-57,-47,-37,-28,-22,-20,-21,-26,-34,-44,-54,-63,-63,-57,-47,-37,-28,-22,-20,-21,-26,-34,-44,-54,-63,-63,-57,-47,-37,-28,-22,-20,-21,-26,-34,-41.5,-41.5];
      | D=[190,160,150,140,130,123,110,100,90,80,50,50,49,44,37,31,25,21,20,21,24,24,28,30,29,26,20,14,7,2,-2,-4,-3,1,1,4,6,6,2,-3,-9,-16,-22,-25,-27,-26,-22,-22,-19,-17,-18,-21,-26,-33,-39,-45,-49,-50,-70];
      | plot(C,D);
      | 
      | 
      | %load figure -120deg
      | c=1*exp(sqrt(-1)*(-60*pi/180));
      | l=A1+j*B1;
      | m=l*c;
      | E=real(m);F=imag(m);
      | E=E+34.4400;F=F-118.53;
      | plot(E,F);
      | 
      | %load figure +120deg
      | c=1*exp(sqrt(-1)*(60*pi/180));
      | l=A+j*B;
      | m=l*c;
      | G=real(m);
      | H=imag(m);
      | G=G-117.44;H=H-118.5300;
      | plot(G,H);
      | 
      | color('black');
      | port_label('LConn', 1, 'A')
      | port_label('LConn', 2, 'B')
      | port_label('LConn', 3, 'C')
  49-50 4 : powerlib/Elements/Distributed Parameters Line  Phases=3  Frequency=60  Resistance=R_4  Inductance=L_4  Capacitance=C_4  Length=250*ft2km  x1=[438.082381973315 4184.31863980955 4184.78631236162;376.991118430775 376.991118430775 376.991118430775;0.395156193508634 -0.219969889248016 -1.78941620047031]  x2=[438.082452224228 4184.31869265923 4184.78645444208;376.991118430775 376.991118430775 376.991118430775;0.395155744511295 -0.219969930881038 -1.78941623141995]  x3=[0.574188161856225 12.3295627316036 15.6192586025475;376.991118430775 376.991118430775 376.991118430775;0.392608680074257 -0.220283856360353 -1.78986415990734]  x4=[0.577416249577747 12.3372237739166 15.6222402763462;376.991118430775 376.991118430775 376.991118430775;0.39757114527375 -0.219753772358498 -1.78906641892685]  x5=3.13537493203638e-07  V1=ones(3,3)  V2=ones(3,3)  I1=ones(3,3)  I2=ones(3,3)  nHarmo=1  Measurements=None
      settings: SourceProductName=Simscape Electrical
  4Y PQ : Subsystem  mask(Single Phase ZIP Load){Vnom=1.0*2401.78, fnom=60, Pnom=40e3*a, Qnom=20e3*a, LoadType=constant P, Vlim=0.7}
      mask prompts: Vnom "Nominal Voltage Vn (Vrms)"; fnom "Nominal Frequency fn (Hz)"; Pnom "Nominal Active power (W)"; Qnom "Nominal Reactive power (VAR)"; LoadType "Load Type"; Vlim "Minimum voltage (pu)"
      mask help:
      | Notes:
      | Single Phase ZIP load model which gets converted to constant Z type if the voltage becomes lower than the Minimum Voltage.
      mask TypeOptions LoadType: Constant Z | constant I | constant P
      mask DialogControl ParameterTabVar0 Prompt: Parameters
      mask DialogControl ParameterTabVar1 Prompt: Type
      mask Display:
      | color('red');
      | A=[-210,-180,-170,-160,-147,-140,-130,-120,-110,-80,-50,-49,-45,-39,-33,-26,-21,-18,-17,-19,-22,-22,-26,-27,-25,-22,-16,-9,-3,2,6,6,4,1,1,-3,-4,-2,2,7,14,20,26,29,30,28,24,24,21,20,21,25,31,37,44,49,50,50,80];
      | B=[-41.5,-41.5,-63,-20,-63,-20,-63,-20,-41.5,-41.5,-41.5,-34,-26,-21,-20,-22,-28,-37,-47,-57,-63,-63,-54,-44,-34,-26,-21,-20,-22,-28,-37,-47,-57,-63,-63,-54,-44,-34,-26,-21,-20,-22,-28,-37,-47,-57,-63,-63,-54,-44,-34,-26,-21,-20,-22,-28,-37,-41.50,-41.5];
      | plot(A,B);
      | color('black');
      | port_label('LConn', 1, '+')
  5 : Subsystem
  5 Y I : Subsystem  mask(Single Phase ZIP Load){Vnom=1.0*2401.78, fnom=60, Pnom=20e3*a, Qnom=10e3*a, LoadType=constant I, Vlim=0.7}
      mask prompts: Vnom "Nominal Voltage Vn (Vrms)"; fnom "Nominal Frequency fn (Hz)"; Pnom "Nominal Active power (W)"; Qnom "Nominal Reactive power (VAR)"; LoadType "Load Type"; Vlim "Minimum voltage (pu)"
      mask help:
      | Notes:
      | Single Phase ZIP load model which gets converted to constant Z type if the voltage becomes lower than the Minimum Voltage.
      mask TypeOptions LoadType: Constant Z | constant I | constant P
      mask DialogControl ParameterTabVar0 Prompt: Parameters
      mask DialogControl ParameterTabVar1 Prompt: Type
      mask Display:
      | color('red');
      | A=[-210,-180,-170,-160,-147,-140,-130,-120,-110,-80,-50,-49,-45,-39,-33,-26,-21,-18,-17,-19,-22,-22,-26,-27,-25,-22,-16,-9,-3,2,6,6,4,1,1,-3,-4,-2,2,7,14,20,26,29,30,28,24,24,21,20,21,25,31,37,44,49,50,50,80];
      | B=[-41.5,-41.5,-63,-20,-63,-20,-63,-20,-41.5,-41.5,-41.5,-34,-26,-21,-20,-22,-28,-37,-47,-57,-63,-63,-54,-44,-34,-26,-21,-20,-22,-28,-37,-47,-57,-63,-63,-54,-44,-34,-26,-21,-20,-22,-28,-37,-47,-57,-63,-63,-54,-44,-34,-26,-21,-20,-22,-28,-37,-41.50,-41.5];
      | plot(A,B);
      | color('black');
      | port_label('LConn', 1, '+')
  5-6 11 : powerlib/Elements/Distributed Parameters Line  Phases=1  Frequency=60  Resistance=R_11(3,3)  Inductance=L_11(3,3)  Capacitance=C_11(3,3)  Length=250*ft2km  x1=[3404.23135167358;376.991118430775;2.09338296152756]  x2=[3404.23116066393;376.991118430775;2.09338289099174]  x3=[6.23039399487055;376.991118430775;2.0932660501659]  x4=[6.23720167259854;376.991118430775;2.09338289099487]  x5=3.09938851618982e-07  V1=[2.049e+04;377;-2.115]  V2=[2.048e+04;377;-2.115]  I1=[33.62;377;-2.106]  I2=[35.2;377;-2.126]  nHarmo=1  Measurements=None
      settings: SourceProductName=Simscape Electrical
  50 : powerlib/Measurements/Three-Phase V-I Measurement  VoltageMeasurement=phase-to-ground  SetLabelV=on  LabelV=V50  Vpu=off  VpuLL=off  CurrentMeasurement=no  SetLabelI=on  LabelI=I800  Ipu=off  Pbase=100e6  Vbase=24900  OutputType=Complex  PhasorSimulation=on  PSBequivalent=0
      settings: SourceProductName=Simscape Electrical
  50 Y PQ : Subsystem  mask(Single Phase ZIP Load){Vnom=1.0*2401.78, fnom=60, Pnom=40e3*a, Qnom=20e3*a, LoadType=constant P, Vlim=0.7}
      mask prompts: Vnom "Nominal Voltage Vn (Vrms)"; fnom "Nominal Frequency fn (Hz)"; Pnom "Nominal Active power (W)"; Qnom "Nominal Reactive power (VAR)"; LoadType "Load Type"; Vlim "Minimum voltage (pu)"
      mask help:
      | Notes:
      | Single Phase ZIP load model which gets converted to constant Z type if the voltage becomes lower than the Minimum Voltage.
      mask TypeOptions LoadType: Constant Z | constant I | constant P
      mask DialogControl ParameterTabVar0 Prompt: Parameters
      mask DialogControl ParameterTabVar1 Prompt: Type
      mask Display:
      | color('red');
      | A=[-210,-180,-170,-160,-147,-140,-130,-120,-110,-80,-50,-49,-45,-39,-33,-26,-21,-18,-17,-19,-22,-22,-26,-27,-25,-22,-16,-9,-3,2,6,6,4,1,1,-3,-4,-2,2,7,14,20,26,29,30,28,24,24,21,20,21,25,31,37,44,49,50,50,80];
      | B=[-41.5,-41.5,-63,-20,-63,-20,-63,-20,-41.5,-41.5,-41.5,-34,-26,-21,-20,-22,-28,-37,-47,-57,-63,-63,-54,-44,-34,-26,-21,-20,-22,-28,-37,-47,-57,-63,-63,-54,-44,-34,-26,-21,-20,-22,-28,-37,-47,-57,-63,-63,-54,-44,-34,-26,-21,-20,-22,-28,-37,-41.50,-41.5];
      | plot(A,B);
      | color('black');
      | port_label('LConn', 1, '+')
  50-51 4 : powerlib/Elements/Distributed Parameters Line  Phases=3  Frequency=60  Resistance=R_4  Inductance=L_4  Capacitance=C_4  Length=250*ft2km  x1=[438.082452224228 4184.31869265923 4184.78645444208;376.991118430775 376.991118430775 376.991118430775;0.395155744511295 -0.219969930881038 -1.78941623141995]  x2=[438.082329484253 4184.31877587603 4184.78654270281;376.991118430775 376.991118430775 376.991118430775;0.39515541271065 -0.21996996261785 -1.78941624352335]  x3=[0.57393686554662 12.3309489557381 15.6206924781478;376.991118430775 376.991118430775 376.991118430775;0.39617164859116 -0.220309098310844 -1.7896823279481]  x4=[0.577664593327187 12.3358381236221 15.6208055112394;376.991118430775 376.991118430775 376.991118430775;0.394028244539757 -0.219728554212249 -1.7892482193748]  x5=3.13537493203638e-07  V1=ones(3,3)  V2=ones(3,3)  I1=ones(3,3)  I2=ones(3,3)  nHarmo=1  Measurements=None
      settings: SourceProductName=Simscape Electrical
  51 : powerlib/Measurements/Three-Phase V-I Measurement  VoltageMeasurement=phase-to-ground  SetLabelV=on  LabelV=V51  Vpu=off  VpuLL=off  CurrentMeasurement=no  SetLabelI=on  LabelI=I800  Ipu=off  Pbase=100e6  Vbase=24900  OutputType=Complex  PhasorSimulation=on  PSBequivalent=0
      settings: SourceProductName=Simscape Electrical
  51 Y PQ : Subsystem  mask(Single Phase ZIP Load){Vnom=1.0*2401.78, fnom=60, Pnom=20e3*a, Qnom=10e3*a, LoadType=constant P, Vlim=0.7}
      mask prompts: Vnom "Nominal Voltage Vn (Vrms)"; fnom "Nominal Frequency fn (Hz)"; Pnom "Nominal Active power (W)"; Qnom "Nominal Reactive power (VAR)"; LoadType "Load Type"; Vlim "Minimum voltage (pu)"
      mask help:
      | Notes:
      | Single Phase ZIP load model which gets converted to constant Z type if the voltage becomes lower than the Minimum Voltage.
      mask TypeOptions LoadType: Constant Z | constant I | constant P
      mask DialogControl ParameterTabVar0 Prompt: Parameters
      mask DialogControl ParameterTabVar1 Prompt: Type
      mask Display:
      | color('red');
      | A=[-210,-180,-170,-160,-147,-140,-130,-120,-110,-80,-50,-49,-45,-39,-33,-26,-21,-18,-17,-19,-22,-22,-26,-27,-25,-22,-16,-9,-3,2,6,6,4,1,1,-3,-4,-2,2,7,14,20,26,29,30,28,24,24,21,20,21,25,31,37,44,49,50,50,80];
      | B=[-41.5,-41.5,-63,-20,-63,-20,-63,-20,-41.5,-41.5,-41.5,-34,-26,-21,-20,-22,-28,-37,-47,-57,-63,-63,-54,-44,-34,-26,-21,-20,-22,-28,-37,-47,-57,-63,-63,-54,-44,-34,-26,-21,-20,-22,-28,-37,-47,-57,-63,-63,-54,-44,-34,-26,-21,-20,-22,-28,-37,-41.50,-41.5];
      | plot(A,B);
      | color('black');
      | port_label('LConn', 1, '+')
  51-151 4 : powerlib/Elements/Distributed Parameters Line  Phases=3  Frequency=60  Resistance=R_4  Inductance=L_4  Capacitance=C_4  Length=500*ft2km  x1=[438.082329484253 4184.31877587603 4184.78654270281;376.991118430775 376.991118430775 376.991118430775;0.395037211860418 -0.220067605534543 -1.78951431300311]  x2=[438.082341520395 4184.31885864354 4184.7866258054;376.991118430775 376.991118430775 376.991118430775;0.395037200355283 -0.220067613217667 -1.78951432323398]  x3=[0.575778842174141 12.3330496207326 15.6201594927734;376.991118430775 376.991118430775 376.991118430775;0.394802079099169 -0.220264740200025 -1.78971206009045]  x4=[0.575780868336906 12.3329479343698 15.6200704551699;376.991118430775 376.991118430775 376.991118430775;0.395035925388276 -0.220065767730927 -1.78951271984702]  x5=6.27074986407277e-07  V1=ones(3,3)  V2=ones(3,3)  I1=ones(3,3)  I2=ones(3,3)  nHarmo=1  Measurements=None
      settings: SourceProductName=Simscape Electrical
  52 : powerlib/Measurements/Three-Phase V-I Measurement  VoltageMeasurement=phase-to-ground  SetLabelV=on  LabelV=V52  Vpu=off  VpuLL=off  CurrentMeasurement=no  SetLabelI=on  LabelI=I65  Ipu=off  Pbase=100e6  Vbase=24900  OutputType=Complex  PhasorSimulation=on  PSBequivalent=0
      settings: SourceProductName=Simscape Electrical
  52 Y PQ : Subsystem  mask(Single Phase ZIP Load){Vnom=1.0*2401.78, fnom=60, Pnom=40e3*a, Qnom=20e3*a, LoadType=constant P, Vlim=0.7}
      mask prompts: Vnom "Nominal Voltage Vn (Vrms)"; fnom "Nominal Frequency fn (Hz)"; Pnom "Nominal Active power (W)"; Qnom "Nominal Reactive power (VAR)"; LoadType "Load Type"; Vlim "Minimum voltage (pu)"
      mask help:
      | Notes:
      | Single Phase ZIP load model which gets converted to constant Z type if the voltage becomes lower than the Minimum Voltage.
      mask TypeOptions LoadType: Constant Z | constant I | constant P
      mask DialogControl ParameterTabVar0 Prompt: Parameters
      mask DialogControl ParameterTabVar1 Prompt: Type
      mask Display:
      | color('red');
      | A=[-210,-180,-170,-160,-147,-140,-130,-120,-110,-80,-50,-49,-45,-39,-33,-26,-21,-18,-17,-19,-22,-22,-26,-27,-25,-22,-16,-9,-3,2,6,6,4,1,1,-3,-4,-2,2,7,14,20,26,29,30,28,24,24,21,20,21,25,31,37,44,49,50,50,80];
      | B=[-41.5,-41.5,-63,-20,-63,-20,-63,-20,-41.5,-41.5,-41.5,-34,-26,-21,-20,-22,-28,-37,-47,-57,-63,-63,-54,-44,-34,-26,-21,-20,-22,-28,-37,-47,-57,-63,-63,-54,-44,-34,-26,-21,-20,-22,-28,-37,-47,-57,-63,-63,-54,-44,-34,-26,-21,-20,-22,-28,-37,-41.50,-41.5];
      | plot(A,B);
      | color('black');
      | port_label('LConn', 1, '+')
  52-53 1 : powerlib/Elements/Distributed Parameters Line  Phases=3  Frequency=60  Resistance=R_1  Inductance=L_1  Capacitance=C_1  Length=200*ft2km  x1=[437.848330578358 4190.48566193662 4196.1402512421;376.991118430775 376.991118430775 376.991118430775;1.68953331311643 -2.40624894656862 2.30612137509255]  x2=[438.024054080782 4194.35485073971 4201.03349436917;376.991118430775 376.991118430775 376.991118430775;1.68927111480438 -2.40677184832523 2.30560126488885]  x3=[2.65580208601384 185.726277857161 185.595942736975;376.991118430775 376.991118430775 376.991118430775;0.135453097425512 2.37902431938449 0.793901471371211]  x4=[2.87668218878156 186.074638691771 185.78984682758;376.991118430775 376.991118430775 376.991118430775;2.86538192890159 -0.931120329144322 -2.4810762327301]  x5=2.50829994562911e-07  V1=ones(3,3)  V2=ones(3,3)  I1=ones(3,3)  I2=ones(3,3)  nHarmo=1  Measurements=None
      settings: SourceProductName=Simscape Electrical
  53 : powerlib/Measurements/Three-Phase V-I Measurement  VoltageMeasurement=phase-to-ground  SetLabelV=on  LabelV=V53  Vpu=off  VpuLL=off  CurrentMeasurement=no  SetLabelI=on  LabelI=I65  Ipu=off  Pbase=100e6  Vbase=24900  OutputType=Complex  PhasorSimulation=on  PSBequivalent=0
      settings: SourceProductName=Simscape Electrical
  53 Y PQ : Subsystem  mask(Single Phase ZIP Load){Vnom=1.0*2401.78, fnom=60, Pnom=40e3*a, Qnom=20e3*a, LoadType=constant P, Vlim=0.7}
      mask prompts: Vnom "Nominal Voltage Vn (Vrms)"; fnom "Nominal Frequency fn (Hz)"; Pnom "Nominal Active power (W)"; Qnom "Nominal Reactive power (VAR)"; LoadType "Load Type"; Vlim "Minimum voltage (pu)"
      mask help:
      | Notes:
      | Single Phase ZIP load model which gets converted to constant Z type if the voltage becomes lower than the Minimum Voltage.
      mask TypeOptions LoadType: Constant Z | constant I | constant P
      mask DialogControl ParameterTabVar0 Prompt: Parameters
      mask DialogControl ParameterTabVar1 Prompt: Type
      mask Display:
      | color('red');
      | A=[-210,-180,-170,-160,-147,-140,-130,-120,-110,-80,-50,-49,-45,-39,-33,-26,-21,-18,-17,-19,-22,-22,-26,-27,-25,-22,-16,-9,-3,2,6,6,4,1,1,-3,-4,-2,2,7,14,20,26,29,30,28,24,24,21,20,21,25,31,37,44,49,50,50,80];
      | B=[-41.5,-41.5,-63,-20,-63,-20,-63,-20,-41.5,-41.5,-41.5,-34,-26,-21,-20,-22,-28,-37,-47,-57,-63,-63,-54,-44,-34,-26,-21,-20,-22,-28,-37,-47,-57,-63,-63,-54,-44,-34,-26,-21,-20,-22,-28,-37,-47,-57,-63,-63,-54,-44,-34,-26,-21,-20,-22,-28,-37,-41.50,-41.5];
      | plot(A,B);
      | color('black');
      | port_label('LConn', 1, '+')
  53-54 1 : powerlib/Elements/Distributed Parameters Line  Phases=3  Frequency=60  Resistance=R_1  Inductance=L_1  Capacitance=C_1  Length=125*ft2km  x1=[438.024054080782 4194.35485073971 4201.03349436917;376.991118430775 376.991118430775 376.991118430775;1.68930657505945 -2.40674242748131 2.30563055776386]  x2=[438.133979265469 4196.77368982038 4204.09231927321;376.991118430775 376.991118430775 376.991118430775;1.68914270280172 -2.40706874745299 2.30530611321823]  x3=[2.6578996040819 185.737199338082 185.602010665182;376.991118430775 376.991118430775 376.991118430775;0.135470035460688 2.37913609540494 0.794014798185202]  x4=[2.87856570804437 186.072331578379 185.785479922767;376.991118430775 376.991118430775 376.991118430775;2.8655389008771 -0.931134190230305 -2.48109051710921]  x5=1.56768746601819e-07  V1=ones(3,3)  V2=ones(3,3)  I1=ones(3,3)  I2=ones(3,3)  nHarmo=1  Measurements=None
      settings: SourceProductName=Simscape Electrical
  54 : powerlib/Measurements/Three-Phase V-I Measurement  VoltageMeasurement=phase-to-ground  SetLabelV=on  LabelV=V54  Vpu=off  VpuLL=off  CurrentMeasurement=no  SetLabelI=on  LabelI=I65  Ipu=off  Pbase=100e6  Vbase=24900  OutputType=Complex  PhasorSimulation=on  PSBequivalent=0
      settings: SourceProductName=Simscape Electrical
